simulink library "halin"  (R2021b)
settings: Solver=VariableStepAuto  StartTime=0.0  StopTime=10.0  RelTol=1e-3
undefined symbols (not defined in the file): KHAL_CAN1ABM1E2E_flg, KHAL_CAN1EPB1E2E_flg, KHAL_CAN1EPS1E2E_flg, KHAL_CAN1ESC1E2E_flg, KHAL_CAN1ESC5E2E_flg, KHAL_CAN3BMS1E2E_flg, KHAL_CAN3BMS6E2E_flg, KHAL_CAN3CCU1E2E_flg, KHAL_CAN3CCU2E2E_flg, KHAL_CAN3MCUBF1E2E_flg, KHAL_CAN3MCUBR1E2E_flg, KHAL_CAN3MCUNF1E2E_flg, KHAL_CAN3MCUNR1E2E_flg, KHAL_CAN3Shifter1E2E_flg, KHAL_CAN3Shifter2E2E_flg, KHAL_CAN6FCM2E2E_flg, KHAL_CAN6FCM4E2E_flg, TRUE
libraries: simulink x791, FVT_lib x214, hcu_lib x58
(part 3 of 25)

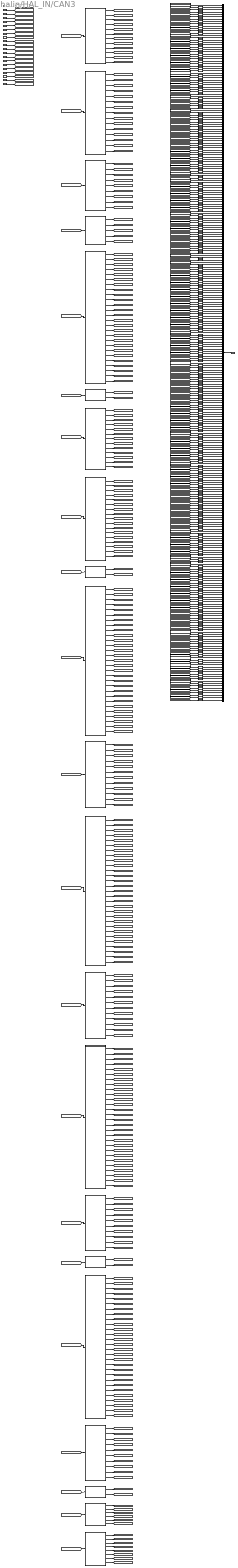
== system halin/HAL_IN/CAN3 ==
  DT_CAN3_SG_BMS1 : Inport
  DT_CAN3_SG_BMS3 : Inport  Port=2
  DT_CAN3_SG_BMS4 : Inport  Port=3
  DT_CAN3_SG_BMS5 : Inport  Port=4
  DT_CAN3_SG_BMS6 : Inport  Port=5
  DT_CAN3_SG_BMS8 : Inport  Port=6
  DT_CAN3_SG_CCU1 : Inport  Port=7
  DT_CAN3_SG_CCU2 : Inport  Port=8
  DT_CAN3_SG_EBM1 : Inport  Port=9
  DT_CAN3_SG_MCU_B_F1 : Inport  Port=10
  DT_CAN3_SG_MCU_B_F2 : Inport  Port=11
  DT_CAN3_SG_MCU_B_R1 : Inport  Port=12
  DT_CAN3_SG_MCU_B_R2 : Inport  Port=13
  DT_CAN3_SG_MCU_N_F1 : Inport  Port=14
  DT_CAN3_SG_MCU_N_F2 : Inport  Port=15
  DT_CAN3_SG_MCU_N_F3 : Inport  Port=16
  DT_CAN3_SG_MCU_N_R1 : Inport  Port=17
  DT_CAN3_SG_MCU_N_R2 : Inport  Port=18
  DT_CAN3_SG_MCU_N_R3 : Inport  Port=19
  DT_CAN3_SG_Shifter1 : Inport  Port=20
  DT_CAN3_SG_Shifter2 : Inport  Port=21
  BMS1 : Subsystem
  BMS3 : Subsystem
  BMS4 : Subsystem
  BMS5 : Subsystem
  BMS6 : Subsystem
  BMS8 : Subsystem
  CCU1 : Subsystem
  CCU2 : Subsystem
  EBM1 : Subsystem
  MCU_B_F1 : Subsystem
  MCU_B_F2 : Subsystem
  MCU_B_R1 : Subsystem
  MCU_B_R2 : Subsystem
  MCU_N_F1 : Subsystem
  MCU_N_F2 : Subsystem
  MCU_N_F3 : Subsystem
  MCU_N_R1 : Subsystem
  MCU_N_R2 : Subsystem
  MCU_N_R3 : Subsystem
  Shifter1 : Subsystem
  Shifter2 : Subsystem
  UnitConverter{,1,13,22,41..42,45..53,59..61,65,69..70,80,82..83,85,87,91,93..94,101..105,114..115,117..119,142..143,146..148,157..158,160..162,183..187,196..197,199..201,223..224,226..228,237..238,240..242,263..264,269..271,274} (75 alike) : DataTypeConversion  OutDataTypeStr=boolean
  UnitConverter{4..12,14..21,23..31,36..40,72..75,77..78,88..90,95,106,108,111..113,121..127,129..130,135..136,145,149,151,154..156,164..170,172,177..178,188,190,193..195,203..209,211..212,217..218,229,231,234..236,244..252,257..258} (105 alike) : DataTypeConversion  OutDataTypeStr=single
  UnitConverter{2..3,32..35,43..44,54..58,62..64,66..68,71,76,79,81,84,86,92,96..100,107,109..110,116,120,128,131..134,137,140..141,144,150,152..153,159,163,171,173..176,181..182,189,191..192,198,202,210,213..216,219..220,225,230,232..233,239,243,253..256,259..260,265..268,272..273,275..276} (89 alike) : DataTypeConversion  OutDataTypeStr=uint8
  UnitConverter{138..139,179..180,221..222,261..262} (8 alike) : DataTypeConversion  OutDataTypeStr=uint16
  VHAL_CANMsgInvalidBMS1_flg : Subsystem  AncestorBlock=FVT_lib/hal/MsgTimeoutJudge_CAN_AUTOSAR
      mask help: MeasumentTrigerEvent
      mask Display: fprintf('MsgTimeoutJudge_CAN\nAUTOSAR');
  VHAL_CANMsgInvalidBMS3_flg : Subsystem  AncestorBlock=FVT_lib/hal/MsgTimeoutJudge_CAN_AUTOSAR
      mask help: MeasumentTrigerEvent
      mask Display: fprintf('MsgTimeoutJudge_CAN\nAUTOSAR');
  VHAL_CANMsgInvalidBMS4_flg : Subsystem  AncestorBlock=FVT_lib/hal/MsgTimeoutJudge_CAN_AUTOSAR
      mask help: MeasumentTrigerEvent
      mask Display: fprintf('MsgTimeoutJudge_CAN\nAUTOSAR');
  VHAL_CANMsgInvalidBMS5_flg : Subsystem  AncestorBlock=FVT_lib/hal/MsgTimeoutJudge_CAN_AUTOSAR
      mask help: MeasumentTrigerEvent
      mask Display: fprintf('MsgTimeoutJudge_CAN\nAUTOSAR');
  VHAL_CANMsgInvalidBMS6_flg : Subsystem  AncestorBlock=FVT_lib/hal/MsgTimeoutJudge_CAN_AUTOSAR
      mask help: MeasumentTrigerEvent
      mask Display: fprintf('MsgTimeoutJudge_CAN\nAUTOSAR');
  VHAL_CANMsgInvalidBMS8_flg : Subsystem  AncestorBlock=FVT_lib/hal/MsgTimeoutJudge_CAN_AUTOSAR
      mask help: MeasumentTrigerEvent
      mask Display: fprintf('MsgTimeoutJudge_CAN\nAUTOSAR');
  VHAL_CANMsgInvalidCCU1_flg : Subsystem  AncestorBlock=FVT_lib/hal/MsgTimeoutJudge_CAN_AUTOSAR
      mask help: MeasumentTrigerEvent
      mask Display: fprintf('MsgTimeoutJudge_CAN\nAUTOSAR');
  VHAL_CANMsgInvalidCCU2_flg : Subsystem  AncestorBlock=FVT_lib/hal/MsgTimeoutJudge_CAN_AUTOSAR
      mask help: MeasumentTrigerEvent
      mask Display: fprintf('MsgTimeoutJudge_CAN\nAUTOSAR');
  VHAL_CANMsgInvalidEBM1_flg : Subsystem  AncestorBlock=FVT_lib/hal/MsgTimeoutJudge_CAN_AUTOSAR
      mask help: MeasumentTrigerEvent
      mask Display: fprintf('MsgTimeoutJudge_CAN\nAUTOSAR');
  VHAL_CANMsgInvalidMCUBF1_flg : Subsystem  AncestorBlock=FVT_lib/hal/MsgTimeoutJudge_CAN_AUTOSAR
      mask help: MeasumentTrigerEvent
      mask Display: fprintf('MsgTimeoutJudge_CAN\nAUTOSAR');
  VHAL_CANMsgInvalidMCUBF2_flg : Subsystem  AncestorBlock=FVT_lib/hal/MsgTimeoutJudge_CAN_AUTOSAR
      mask help: MeasumentTrigerEvent
      mask Display: fprintf('MsgTimeoutJudge_CAN\nAUTOSAR');
  VHAL_CANMsgInvalidMCUBR1_flg : Subsystem  AncestorBlock=FVT_lib/hal/MsgTimeoutJudge_CAN_AUTOSAR
      mask help: MeasumentTrigerEvent
      mask Display: fprintf('MsgTimeoutJudge_CAN\nAUTOSAR');
  VHAL_CANMsgInvalidMCUBR2_flg : Subsystem  AncestorBlock=FVT_lib/hal/MsgTimeoutJudge_CAN_AUTOSAR
      mask help: MeasumentTrigerEvent
      mask Display: fprintf('MsgTimeoutJudge_CAN\nAUTOSAR');
  VHAL_CANMsgInvalidMCUNF1_flg : Subsystem  AncestorBlock=FVT_lib/hal/MsgTimeoutJudge_CAN_AUTOSAR
      mask help: MeasumentTrigerEvent
      mask Display: fprintf('MsgTimeoutJudge_CAN\nAUTOSAR');
  VHAL_CANMsgInvalidMCUNF2_flg : Subsystem  AncestorBlock=FVT_lib/hal/MsgTimeoutJudge_CAN_AUTOSAR
      mask help: MeasumentTrigerEvent
      mask Display: fprintf('MsgTimeoutJudge_CAN\nAUTOSAR');
  VHAL_CANMsgInvalidMCUNF3_flg : Subsystem  AncestorBlock=FVT_lib/hal/MsgTimeoutJudge_CAN_AUTOSAR
      mask help: MeasumentTrigerEvent
      mask Display: fprintf('MsgTimeoutJudge_CAN\nAUTOSAR');
  VHAL_CANMsgInvalidMCUNR1_flg : Subsystem  AncestorBlock=FVT_lib/hal/MsgTimeoutJudge_CAN_AUTOSAR
      mask help: MeasumentTrigerEvent
      mask Display: fprintf('MsgTimeoutJudge_CAN\nAUTOSAR');
  VHAL_CANMsgInvalidMCUNR2_flg : Subsystem  AncestorBlock=FVT_lib/hal/MsgTimeoutJudge_CAN_AUTOSAR
      mask help: MeasumentTrigerEvent
      mask Display: fprintf('MsgTimeoutJudge_CAN\nAUTOSAR');
  VHAL_CANMsgInvalidMCUNR3_flg : Subsystem  AncestorBlock=FVT_lib/hal/MsgTimeoutJudge_CAN_AUTOSAR
      mask help: MeasumentTrigerEvent
      mask Display: fprintf('MsgTimeoutJudge_CAN\nAUTOSAR');
  VHAL_CANMsgInvalidShifter1_flg : Subsystem  AncestorBlock=FVT_lib/hal/MsgTimeoutJudge_CAN_AUTOSAR
      mask help: MeasumentTrigerEvent
      mask Display: fprintf('MsgTimeoutJudge_CAN\nAUTOSAR');
  VHAL_CANMsgInvalidShifter2_flg : Subsystem  AncestorBlock=FVT_lib/hal/MsgTimeoutJudge_CAN_AUTOSAR
      mask help: MeasumentTrigerEvent
      mask Display: fprintf('MsgTimeoutJudge_CAN\nAUTOSAR');
  bus_creator : BusCreator  Inputs=298  OutDataTypeStr=Bus: BHAL_CAN3_outputs  NonVirtualBus=on
  HAL_CAN3_outputs : Outport
  wires:
  DT_CAN3_SG_BMS1/1 -> [DT_CAN3_SG_BMS1]
  DT_CAN3_SG_BMS3/1 -> [DT_CAN3_SG_BMS3]
  DT_CAN3_SG_BMS4/1 -> [DT_CAN3_SG_BMS4]
  DT_CAN3_SG_BMS5/1 -> [DT_CAN3_SG_BMS5]
  DT_CAN3_SG_BMS6/1 -> [DT_CAN3_SG_BMS6]
  DT_CAN3_SG_BMS8/1 -> [DT_CAN3_SG_BMS8]
  DT_CAN3_SG_CCU1/1 -> [DT_CAN3_SG_CCU1]
  DT_CAN3_SG_CCU2/1 -> [DT_CAN3_SG_CCU2]
  DT_CAN3_SG_EBM1/1 -> [DT_CAN3_SG_EBM1]
  DT_CAN3_SG_MCU_B_F1/1 -> [DT_CAN3_SG_MCU_B_F1]
  DT_CAN3_SG_MCU_B_F2/1 -> [DT_CAN3_SG_MCU_B_F2]
  DT_CAN3_SG_MCU_B_R1/1 -> [DT_CAN3_SG_MCU_B_R1]
  DT_CAN3_SG_MCU_B_R2/1 -> [DT_CAN3_SG_MCU_B_R2]
  DT_CAN3_SG_MCU_N_F1/1 -> [DT_CAN3_SG_MCU_N_F1]
  DT_CAN3_SG_MCU_N_F2/1 -> [DT_CAN3_SG_MCU_N_F2]
  DT_CAN3_SG_MCU_N_F3/1 -> [DT_CAN3_SG_MCU_N_F3]
  DT_CAN3_SG_MCU_N_R1/1 -> [DT_CAN3_SG_MCU_N_R1]
  DT_CAN3_SG_MCU_N_R2/1 -> [DT_CAN3_SG_MCU_N_R2]
  DT_CAN3_SG_MCU_N_R3/1 -> [DT_CAN3_SG_MCU_N_R3]
  DT_CAN3_SG_Shifter1/1 -> [DT_CAN3_SG_Shifter1]
  DT_CAN3_SG_Shifter2/1 -> [DT_CAN3_SG_Shifter2]
  [DT_CAN3_SG_BMS1] -> BMS1/1(DT_CAN3_SG_BMS1)
  [DT_CAN3_SG_BMS3] -> BMS3/1(DT_CAN3_SG_BMS3)
  [DT_CAN3_SG_BMS4] -> BMS4/1(DT_CAN3_SG_BMS4)
  [DT_CAN3_SG_BMS5] -> BMS5/1(DT_CAN3_SG_BMS5)
  [DT_CAN3_SG_BMS6] -> BMS6/1(DT_CAN3_SG_BMS6)
  [DT_CAN3_SG_BMS8] -> BMS8/1(DT_CAN3_SG_BMS8)
  [DT_CAN3_SG_CCU1] -> CCU1/1(DT_CAN3_SG_CCU1)
  [DT_CAN3_SG_CCU2] -> CCU2/1(DT_CAN3_SG_CCU2)
  [DT_CAN3_SG_EBM1] -> EBM1/1(DT_CAN3_SG_EBM1)
  [DT_CAN3_SG_MCU_B_F1] -> MCU_B_F1/1(DT_CAN3_SG_MCU_B_F1)
  [DT_CAN3_SG_MCU_B_F2] -> MCU_B_F2/1(DT_CAN3_SG_MCU_B_F2)
  [DT_CAN3_SG_MCU_B_R1] -> MCU_B_R1/1(DT_CAN3_SG_MCU_B_R1)
  [DT_CAN3_SG_MCU_B_R2] -> MCU_B_R2/1(DT_CAN3_SG_MCU_B_R2)
  [DT_CAN3_SG_MCU_N_F1] -> MCU_N_F1/1(DT_CAN3_SG_MCU_N_F1)
  [DT_CAN3_SG_MCU_N_F2] -> MCU_N_F2/1(DT_CAN3_SG_MCU_N_F2)
  [DT_CAN3_SG_MCU_N_F3] -> MCU_N_F3/1(DT_CAN3_SG_MCU_N_F3)
  [DT_CAN3_SG_MCU_N_R1] -> MCU_N_R1/1(DT_CAN3_SG_MCU_N_R1)
  [DT_CAN3_SG_MCU_N_R2] -> MCU_N_R2/1(DT_CAN3_SG_MCU_N_R2)
  [DT_CAN3_SG_MCU_N_R3] -> MCU_N_R3/1(DT_CAN3_SG_MCU_N_R3)
  [DT_CAN3_SG_Shifter1] -> Shifter1/1(DT_CAN3_SG_Shifter1)
  [DT_CAN3_SG_Shifter2] -> Shifter2/1(DT_CAN3_SG_Shifter2)
  bus_creator/1 -> HAL_CAN3_outputs/1
  VHAL_CANMsgInvalidBMS1_flg/1(Out) -> bus_creator/1
  BMS1/1(VHAL_BMS1CSErr_flg) -> [VHAL_BMS1CSErr_flg]
  UnitConverter/1 -> bus_creator/2  "VHAL_BMS1CSErr_flg"
  [VHAL_BMS1CSErr_flg] -> UnitConverter/1
  BMS1/2(VHAL_BMS1RCErr_flg) -> [VHAL_BMS1RCErr_flg]
  UnitConverter1/1 -> bus_creator/3  "VHAL_BMS1RCErr_flg"
  [VHAL_BMS1RCErr_flg] -> UnitConverter1/1
  BMS1/3(VHAL_BMSChckSum1_enum) -> [VHAL_BMSChckSum1_enum]
  UnitConverter2/1 -> bus_creator/4  "VHAL_BMSChckSum1_enum"
  [VHAL_BMSChckSum1_enum] -> UnitConverter2/1
  BMS1/4(VHAL_BMSRolCnct1_enum) -> [VHAL_BMSRolCnct1_enum]
  UnitConverter3/1 -> bus_creator/5  "VHAL_BMSRolCnct1_enum"
  [VHAL_BMSRolCnct1_enum] -> UnitConverter3/1
  BMS1/5(VHAL_HVBPwrAvailChrg_kW) -> [VHAL_HVBPwrAvailChrg_kW]
  UnitConverter4/1 -> bus_creator/6  "VHAL_HVBPwrAvailChrg_kW"
  [VHAL_HVBPwrAvailChrg_kW] -> UnitConverter4/1
  BMS1/6(VHAL_HVBPwrAvailChrg30_kW) -> [VHAL_HVBPwrAvailChrg30_kW]
  UnitConverter5/1 -> bus_creator/7  "VHAL_HVBPwrAvailChrg30_kW"
  [VHAL_HVBPwrAvailChrg30_kW] -> UnitConverter5/1
  BMS1/7(VHAL_HVBPwrAvailChrg60_kW) -> [VHAL_HVBPwrAvailChrg60_kW]
  UnitConverter6/1 -> bus_creator/8  "VHAL_HVBPwrAvailChrg60_kW"
  [VHAL_HVBPwrAvailChrg60_kW] -> UnitConverter6/1
  BMS1/8(VHAL_HVBPwrAvailDchrg_kW) -> [VHAL_HVBPwrAvailDchrg_kW]
  UnitConverter7/1 -> bus_creator/9  "VHAL_HVBPwrAvailDchrg_kW"
  [VHAL_HVBPwrAvailDchrg_kW] -> UnitConverter7/1
  BMS1/9(VHAL_HVBPwrAvailDchrg30_kW) -> [VHAL_HVBPwrAvailDchrg30_kW]
  UnitConverter8/1 -> bus_creator/10  "VHAL_HVBPwrAvailDchrg30_kW"
  [VHAL_HVBPwrAvailDchrg30_kW] -> UnitConverter8/1
  BMS1/10(VHAL_HVBPwrAvailDchrg60_kW) -> [VHAL_HVBPwrAvailDchrg60_kW]
  UnitConverter9/1 -> bus_creator/11  "VHAL_HVBPwrAvailDchrg60_kW"
  [VHAL_HVBPwrAvailDchrg60_kW] -> UnitConverter9/1
  BMS1/11(VHAL_HVBattCurr_A) -> [VHAL_HVBattCurr_A]
  UnitConverter10/1 -> bus_creator/12  "VHAL_HVBattCurr_A"
  [VHAL_HVBattCurr_A] -> UnitConverter10/1
  BMS1/12(VHAL_HVBattVolt_V) -> [VHAL_HVBattVolt_V]
  UnitConverter11/1 -> bus_creator/13  "VHAL_HVBattVolt_V"
  [VHAL_HVBattVolt_V] -> UnitConverter11/1
  VHAL_CANMsgInvalidBMS3_flg/1(Out) -> bus_creator/14
  BMS3/1(VHAL_ACChrgCurrDis_A) -> [VHAL_ACChrgCurrDis_A]
  UnitConverter12/1 -> bus_creator/15  "VHAL_ACChrgCurrDis_A"
  [VHAL_ACChrgCurrDis_A] -> UnitConverter12/1
  BMS3/2(VHAL_FireDetErr_flg) -> [VHAL_FireDetErr_flg]
  UnitConverter13/1 -> bus_creator/16  "VHAL_FireDetErr_flg"
  [VHAL_FireDetErr_flg] -> UnitConverter13/1
  BMS3/3(VHAL_HVBChrgPwr_kWh) -> [VHAL_HVBChrgPwr_kWh]
  UnitConverter14/1 -> bus_creator/17  "VHAL_HVBChrgPwr_kWh"
  [VHAL_HVBChrgPwr_kWh] -> UnitConverter14/1
  BMS3/4(VHAL_HVBChrgPwrTotal_kWh) -> [VHAL_HVBChrgPwrTotal_kWh]
  UnitConverter15/1 -> bus_creator/18  "VHAL_HVBChrgPwrTotal_kWh"
  [VHAL_HVBChrgPwrTotal_kWh] -> UnitConverter15/1
  BMS3/5(VHAL_HVBDrvPwr_kWh) -> [VHAL_HVBDrvPwr_kWh]
  UnitConverter16/1 -> bus_creator/19  "VHAL_HVBDrvPwr_kWh"
  [VHAL_HVBDrvPwr_kWh] -> UnitConverter16/1
  BMS3/6(VHAL_HVBDrvPwrTotal_kWh) -> [VHAL_HVBDrvPwrTotal_kWh]
  UnitConverter17/1 -> bus_creator/20  "VHAL_HVBDrvPwrTotal_kWh"
  [VHAL_HVBDrvPwrTotal_kWh] -> UnitConverter17/1
  BMS3/7(VHAL_HVBFullChrgPwr_kWh) -> [VHAL_HVBFullChrgPwr_kWh]
  UnitConverter18/1 -> bus_creator/21  "VHAL_HVBFullChrgPwr_kWh"
  [VHAL_HVBFullChrgPwr_kWh] -> UnitConverter18/1
  BMS3/8(VHAL_HVBIsoImpedenceN_Megaohm) -> [VHAL_HVBIsoImpedenceN_Megaohm]
  UnitConverter19/1 -> bus_creator/22  "VHAL_HVBIsoImpedenceN_Megaohm"
  [VHAL_HVBIsoImpedenceN_Megaohm] -> UnitConverter19/1
  BMS3/9(VHAL_HVBIsoImpedenceP_Megaohm) -> [VHAL_HVBIsoImpedenceP_Megaohm]
  UnitConverter20/1 -> bus_creator/23  "VHAL_HVBIsoImpedenceP_Megaohm"
  [VHAL_HVBIsoImpedenceP_Megaohm] -> UnitConverter20/1
  BMS3/10(VHAL_HVBSOH_pct) -> [VHAL_HVBSOH_pct]
  UnitConverter21/1 -> bus_creator/24  "VHAL_HVBSOH_pct"
  [VHAL_HVBSOH_pct] -> UnitConverter21/1
  BMS3/11(VHAL_HVBattErr_flg) -> [VHAL_HVBattErr_flg]
  UnitConverter22/1 -> bus_creator/25  "VHAL_HVBattErr_flg"
  [VHAL_HVBattErr_flg] -> UnitConverter22/1
  BMS3/12(VHAL_HVBattPackVolt_V) -> [VHAL_HVBattPackVolt_V]
  UnitConverter23/1 -> bus_creator/26  "VHAL_HVBattPackVolt_V"
  [VHAL_HVBattPackVolt_V] -> UnitConverter23/1
  BMS3/13(VHAL_HVBattSOC_pct) -> [VHAL_HVBattSOC_pct]
  UnitConverter24/1 -> bus_creator/27  "VHAL_HVBattSOC_pct"
  [VHAL_HVBattSOC_pct] -> UnitConverter24/1
  BMS3/14(VHAL_HVBattSOCDis_pct) -> [VHAL_HVBattSOCDis_pct]
  UnitConverter25/1 -> bus_creator/28  "VHAL_HVBattSOCDis_pct"
  [VHAL_HVBattSOCDis_pct] -> UnitConverter25/1
  BMS3/15(VHAL_RemainChrgTime_min) -> [VHAL_RemainChrgTime_min]
  UnitConverter26/1 -> bus_creator/29  "VHAL_RemainChrgTime_min"
  [VHAL_RemainChrgTime_min] -> UnitConverter26/1
  VHAL_CANMsgInvalidBMS4_flg/1(Out) -> bus_creator/30
  BMS4/1(VHAL_CellTempAvg_C) -> [VHAL_CellTempAvg_C]
  UnitConverter27/1 -> bus_creator/31  "VHAL_CellTempAvg_C"
  [VHAL_CellTempAvg_C] -> UnitConverter27/1
  BMS4/2(VHAL_HVBCellVoltMax_mV) -> [VHAL_HVBCellVoltMax_mV]
  UnitConverter28/1 -> bus_creator/32  "VHAL_HVBCellVoltMax_mV"
  [VHAL_HVBCellVoltMax_mV] -> UnitConverter28/1
  BMS4/3(VHAL_HVBCellVoltMin_mV) -> [VHAL_HVBCellVoltMin_mV]
  UnitConverter29/1 -> bus_creator/33  "VHAL_HVBCellVoltMin_mV"
  [VHAL_HVBCellVoltMin_mV] -> UnitConverter29/1
  BMS4/4(VHAL_HVBMTempMax_C) -> [VHAL_HVBMTempMax_C]
  UnitConverter30/1 -> bus_creator/34  "VHAL_HVBMTempMax_C"
  [VHAL_HVBMTempMax_C] -> UnitConverter30/1
  BMS4/5(VHAL_HVBMTempMin_C) -> [VHAL_HVBMTempMin_C]
  UnitConverter31/1 -> bus_creator/35  "VHAL_HVBMTempMin_C"
  [VHAL_HVBMTempMin_C] -> UnitConverter31/1
  BMS4/6(VHAL_MaxCellTempNum_enum) -> [VHAL_MaxCellTempNum_enum]
  UnitConverter32/1 -> bus_creator/36  "VHAL_MaxCellTempNum_enum"
  [VHAL_MaxCellTempNum_enum] -> UnitConverter32/1
  BMS4/7(VHAL_MaxCellVoltNum_enum) -> [VHAL_MaxCellVoltNum_enum]
  UnitConverter33/1 -> bus_creator/37  "VHAL_MaxCellVoltNum_enum"
  [VHAL_MaxCellVoltNum_enum] -> UnitConverter33/1
  BMS4/8(VHAL_MinCellTempNum_enum) -> [VHAL_MinCellTempNum_enum]
  UnitConverter34/1 -> bus_creator/38  "VHAL_MinCellTempNum_enum"
  [VHAL_MinCellTempNum_enum] -> UnitConverter34/1
  BMS4/9(VHAL_MinCellVoltNum_enum) -> [VHAL_MinCellVoltNum_enum]
  UnitConverter35/1 -> bus_creator/39  "VHAL_MinCellVoltNum_enum"
  [VHAL_MinCellVoltNum_enum] -> UnitConverter35/1
  VHAL_CANMsgInvalidBMS5_flg/1(Out) -> bus_creator/40
  BMS5/1(VHAL_HVInVolt_V) -> [VHAL_HVInVolt_V]
  UnitConverter36/1 -> bus_creator/41  "VHAL_HVInVolt_V"
  [VHAL_HVInVolt_V] -> UnitConverter36/1
  BMS5/2(VHAL_LVBattDet12V_V) -> [VHAL_LVBattDet12V_V]
  UnitConverter37/1 -> bus_creator/42  "VHAL_LVBattDet12V_V"
  [VHAL_LVBattDet12V_V] -> UnitConverter37/1
  BMS5/3(VHAL_OBCACCSLimit_A) -> [VHAL_OBCACCSLimit_A]
  UnitConverter38/1 -> bus_creator/43  "VHAL_OBCACCSLimit_A"
  [VHAL_OBCACCSLimit_A] -> UnitConverter38/1
  BMS5/4(VHAL_OBCDCCurLm_A) -> [VHAL_OBCDCCurLm_A]
  UnitConverter39/1 -> bus_creator/44  "VHAL_OBCDCCurLm_A"
  [VHAL_OBCDCCurLm_A] -> UnitConverter39/1
  BMS5/5(VHAL_OBCDCVoltLm_V) -> [VHAL_OBCDCVoltLm_V]
  UnitConverter40/1 -> bus_creator/45  "VHAL_OBCDCVoltLm_V"
  [VHAL_OBCDCVoltLm_V] -> UnitConverter40/1
  VHAL_CANMsgInvalidBMS6_flg/1(Out) -> bus_creator/46
  BMS6/1(VHAL_BMS6CSErr_flg) -> [VHAL_BMS6CSErr_flg]
  UnitConverter41/1 -> bus_creator/47  "VHAL_BMS6CSErr_flg"
  [VHAL_BMS6CSErr_flg] -> UnitConverter41/1
  BMS6/2(VHAL_BMS6RCErr_flg) -> [VHAL_BMS6RCErr_flg]
  UnitConverter42/1 -> bus_creator/48  "VHAL_BMS6RCErr_flg"
  [VHAL_BMS6RCErr_flg] -> UnitConverter42/1
  BMS6/3(VHAL_BMSChckSum_enum) -> [VHAL_BMSChckSum_enum]
  UnitConverter43/1 -> bus_creator/49  "VHAL_BMSChckSum_enum"
  [VHAL_BMSChckSum_enum] -> UnitConverter43/1
  BMS6/4(VHAL_BMSRolCnct_enum) -> [VHAL_BMSRolCnct_enum]
  UnitConverter44/1 -> bus_creator/50  "VHAL_BMSRolCnct_enum"
  [VHAL_BMSRolCnct_enum] -> UnitConverter44/1
  BMS6/5(VHAL_BMSREADY_flg) -> [VHAL_BMSREADY_flg]
  UnitConverter45/1 -> bus_creator/51  "VHAL_BMSREADY_flg"
  [VHAL_BMSREADY_flg] -> UnitConverter45/1
  BMS6/6(VHAL_BMSWarn1_flg) -> [VHAL_BMSWarn1_flg]
  UnitConverter46/1 -> bus_creator/52  "VHAL_BMSWarn1_flg"
  [VHAL_BMSWarn1_flg] -> UnitConverter46/1
  BMS6/7(VHAL_BMSWarn2_flg) -> [VHAL_BMSWarn2_flg]
  UnitConverter47/1 -> bus_creator/53  "VHAL_BMSWarn2_flg"
  [VHAL_BMSWarn2_flg] -> UnitConverter47/1
  BMS6/8(VHAL_BMSWarn3_flg) -> [VHAL_BMSWarn3_flg]
  UnitConverter48/1 -> bus_creator/54  "VHAL_BMSWarn3_flg"
  [VHAL_BMSWarn3_flg] -> UnitConverter48/1
  BMS6/9(VHAL_BMSWarn4_flg) -> [VHAL_BMSWarn4_flg]
  UnitConverter49/1 -> bus_creator/55  "VHAL_BMSWarn4_flg"
  [VHAL_BMSWarn4_flg] -> UnitConverter49/1
  BMS6/10(VHAL_BMSWarn5_flg) -> [VHAL_BMSWarn5_flg]
  UnitConverter50/1 -> bus_creator/56  "VHAL_BMSWarn5_flg"
  [VHAL_BMSWarn5_flg] -> UnitConverter50/1
  BMS6/11(VHAL_BMSWarn6_flg) -> [VHAL_BMSWarn6_flg]
  UnitConverter51/1 -> bus_creator/57  "VHAL_BMSWarn6_flg"
  [VHAL_BMSWarn6_flg] -> UnitConverter51/1
  BMS6/12(VHAL_BMSWarn7_flg) -> [VHAL_BMSWarn7_flg]
  UnitConverter52/1 -> bus_creator/58  "VHAL_BMSWarn7_flg"
  [VHAL_BMSWarn7_flg] -> UnitConverter52/1
  BMS6/13(VHAL_BMSWarn8_flg) -> [VHAL_BMSWarn8_flg]
  UnitConverter53/1 -> bus_creator/59  "VHAL_BMSWarn8_flg"
  [VHAL_BMSWarn8_flg] -> UnitConverter53/1
  BMS6/14(VHAL_ChrgInLockReq_enum) -> [VHAL_ChrgInLockReq_enum]
  UnitConverter54/1 -> bus_creator/60  "VHAL_ChrgInLockReq_enum"
  [VHAL_ChrgInLockReq_enum] -> UnitConverter54/1
  BMS6/15(VHAL_ChrgPlugSta_enum) -> [VHAL_ChrgPlugSta_enum]
  UnitConverter55/1 -> bus_creator/61  "VHAL_ChrgPlugSta_enum"
  [VHAL_ChrgPlugSta_enum] -> UnitConverter55/1
  BMS6/16(VHAL_DisChrgPlugErr_enum) -> [VHAL_DisChrgPlugErr_enum]
  UnitConverter56/1 -> bus_creator/62  "VHAL_DisChrgPlugErr_enum"
  [VHAL_DisChrgPlugErr_enum] -> UnitConverter56/1
  BMS6/17(VHAL_ExtChrgSta_enum) -> [VHAL_ExtChrgSta_enum]
  UnitConverter57/1 -> bus_creator/63  "VHAL_ExtChrgSta_enum"
  [VHAL_ExtChrgSta_enum] -> UnitConverter57/1
  BMS6/18(VHAL_HVBChrgErr_enum) -> [VHAL_HVBChrgErr_enum]
  UnitConverter58/1 -> bus_creator/64  "VHAL_HVBChrgErr_enum"
  [VHAL_HVBChrgErr_enum] -> UnitConverter58/1
  BMS6/19(VHAL_HVBContactorSta_flg) -> [VHAL_HVBContactorSta_flg]
  UnitConverter59/1 -> bus_creator/65  "VHAL_HVBContactorSta_flg"
  [VHAL_HVBContactorSta_flg] -> UnitConverter59/1
  BMS6/20(VHAL_HVBHVILErr_flg) -> [VHAL_HVBHVILErr_flg]
  UnitConverter60/1 -> bus_creator/66  "VHAL_HVBHVILErr_flg"
  [VHAL_HVBHVILErr_flg] -> UnitConverter60/1
  BMS6/21(VHAL_HVBOvrTempErr_flg) -> [VHAL_HVBOvrTempErr_flg]
  UnitConverter61/1 -> bus_creator/67  "VHAL_HVBOvrTempErr_flg"
  [VHAL_HVBOvrTempErr_flg] -> UnitConverter61/1
  BMS6/22(VHAL_HVBOvrTempWarn_enum) -> [VHAL_HVBOvrTempWarn_enum]
  UnitConverter62/1 -> bus_creator/68  "VHAL_HVBOvrTempWarn_enum"
  [VHAL_HVBOvrTempWarn_enum] -> UnitConverter62/1
  BMS6/23(VHAL_HVBPreheatPrecoolSta_enum) -> [VHAL_HVBPreheatPrecoolSta_enum]
  UnitConverter63/1 -> bus_creator/69  "VHAL_HVBPreheatPrecoolSta_enum"
  [VHAL_HVBPreheatPrecoolSta_enum] -> UnitConverter63/1
  BMS6/24(VHAL_HVBattReady4Pre_enum) -> [VHAL_HVBattReady4Pre_enum]
  UnitConverter64/1 -> bus_creator/70  "VHAL_HVBattReady4Pre_enum"
  [VHAL_HVBattReady4Pre_enum] -> UnitConverter64/1
  BMS6/25(VHAL_HVILSta_flg) -> [VHAL_HVILSta_flg]
  UnitConverter65/1 -> bus_creator/71  "VHAL_HVILSta_flg"
  [VHAL_HVILSta_flg] -> UnitConverter65/1
  BMS6/26(VHAL_V2LSta_enum) -> [VHAL_V2LSta_enum]
  UnitConverter66/1 -> bus_creator/72  "VHAL_V2LSta_enum"
  [VHAL_V2LSta_enum] -> UnitConverter66/1
  VHAL_CANMsgInvalidBMS8_flg/1(Out) -> bus_creator/73
  BMS8/1(VHAL_MainRlyNegSta_enum) -> [VHAL_MainRlyNegSta_enum]
  UnitConverter67/1 -> bus_creator/74  "VHAL_MainRlyNegSta_enum"
  [VHAL_MainRlyNegSta_enum] -> UnitConverter67/1
  BMS8/2(VHAL_MainRlyPosSta_enum) -> [VHAL_MainRlyPosSta_enum]
  UnitConverter68/1 -> bus_creator/75  "VHAL_MainRlyPosSta_enum"
  [VHAL_MainRlyPosSta_enum] -> UnitConverter68/1
  VHAL_CANMsgInvalidCCU1_flg/1(Out) -> bus_creator/76
  CCU1/1(VHAL_CCU1CSErr_flg) -> [VHAL_CCU1CSErr_flg]
  UnitConverter69/1 -> bus_creator/77  "VHAL_CCU1CSErr_flg"
  [VHAL_CCU1CSErr_flg] -> UnitConverter69/1
  CCU1/2(VHAL_CCU1RCErr_flg) -> [VHAL_CCU1RCErr_flg]
  UnitConverter70/1 -> bus_creator/78  "VHAL_CCU1RCErr_flg"
  [VHAL_CCU1RCErr_flg] -> UnitConverter70/1
  CCU1/3(VHAL_CSCCU1_enum) -> [VHAL_CSCCU1_enum]
  UnitConverter71/1 -> bus_creator/79  "VHAL_CSCCU1_enum"
  [VHAL_CSCCU1_enum] -> UnitConverter71/1
  CCU1/4(VHAL_DCDCAuxCur_A) -> [VHAL_DCDCAuxCur_A]
  UnitConverter72/1 -> bus_creator/80  "VHAL_DCDCAuxCur_A"
  [VHAL_DCDCAuxCur_A] -> UnitConverter72/1
  CCU1/5(VHAL_DCDCAuxVolt_V) -> [VHAL_DCDCAuxVolt_V]
  UnitConverter73/1 -> bus_creator/81  "VHAL_DCDCAuxVolt_V"
  [VHAL_DCDCAuxVolt_V] -> UnitConverter73/1
  CCU1/6(VHAL_DCDCHVCur_A) -> [VHAL_DCDCHVCur_A]
  UnitConverter74/1 -> bus_creator/82  "VHAL_DCDCHVCur_A"
  [VHAL_DCDCHVCur_A] -> UnitConverter74/1
  CCU1/7(VHAL_DCDCInVoltInf_V) -> [VHAL_DCDCInVoltInf_V]
  UnitConverter75/1 -> bus_creator/83  "VHAL_DCDCInVoltInf_V"
  [VHAL_DCDCInVoltInf_V] -> UnitConverter75/1
  CCU1/8(VHAL_DCDCPreCompleted_enum) -> [VHAL_DCDCPreCompleted_enum]
  UnitConverter76/1 -> bus_creator/84  "VHAL_DCDCPreCompleted_enum"
  [VHAL_DCDCPreCompleted_enum] -> UnitConverter76/1
  CCU1/9(VHAL_OBCDCCurrInf_A) -> [VHAL_OBCDCCurrInf_A]
  UnitConverter77/1 -> bus_creator/85  "VHAL_OBCDCCurrInf_A"
  [VHAL_OBCDCCurrInf_A] -> UnitConverter77/1
  CCU1/10(VHAL_OBCDCVoltInf_V) -> [VHAL_OBCDCVoltInf_V]
  UnitConverter78/1 -> bus_creator/86  "VHAL_OBCDCVoltInf_V"
  [VHAL_OBCDCVoltInf_V] -> UnitConverter78/1
  CCU1/11(VHAL_OBCPreCompleted_enum) -> [VHAL_OBCPreCompleted_enum]
  UnitConverter79/1 -> bus_creator/87  "VHAL_OBCPreCompleted_enum"
  [VHAL_OBCPreCompleted_enum] -> UnitConverter79/1
  CCU1/12(VHAL_OBCWakeup4Plugin_flg) -> [VHAL_OBCWakeup4Plugin_flg]
  UnitConverter80/1 -> bus_creator/88  "VHAL_OBCWakeup4Plugin_flg"
  [VHAL_OBCWakeup4Plugin_flg] -> UnitConverter80/1
  CCU1/13(VHAL_RCCCU1_enum) -> [VHAL_RCCCU1_enum]
  UnitConverter81/1 -> bus_creator/89  "VHAL_RCCCU1_enum"
  [VHAL_RCCCU1_enum] -> UnitConverter81/1
  VHAL_CANMsgInvalidCCU2_flg/1(Out) -> bus_creator/90
  CCU2/1(VHAL_CCU2CSErr_flg) -> [VHAL_CCU2CSErr_flg]
  UnitConverter82/1 -> bus_creator/91  "VHAL_CCU2CSErr_flg"
  [VHAL_CCU2CSErr_flg] -> UnitConverter82/1
  CCU2/2(VHAL_CCU2RCErr_flg) -> [VHAL_CCU2RCErr_flg]
  UnitConverter83/1 -> bus_creator/92  "VHAL_CCU2RCErr_flg"
  [VHAL_CCU2RCErr_flg] -> UnitConverter83/1
  CCU2/3(VHAL_CSCCU2_enum) -> [VHAL_CSCCU2_enum]
  UnitConverter84/1 -> bus_creator/93  "VHAL_CSCCU2_enum"
  [VHAL_CSCCU2_enum] -> UnitConverter84/1
  CCU2/4(VHAL_DCDCEnaSta_flg) -> [VHAL_DCDCEnaSta_flg]
  UnitConverter85/1 -> bus_creator/94  "VHAL_DCDCEnaSta_flg"
  [VHAL_DCDCEnaSta_flg] -> UnitConverter85/1
  CCU2/5(VHAL_DCDCFaultSta_enum) -> [VHAL_DCDCFaultSta_enum]
  UnitConverter86/1 -> bus_creator/95  "VHAL_DCDCFaultSta_enum"
  [VHAL_DCDCFaultSta_enum] -> UnitConverter86/1
  CCU2/6(VHAL_DCDCReady4Pre_flg) -> [VHAL_DCDCReady4Pre_flg]
  UnitConverter87/1 -> bus_creator/96  "VHAL_DCDCReady4Pre_flg"
  [VHAL_DCDCReady4Pre_flg] -> UnitConverter87/1
  CCU2/7(VHAL_DCDCTemp_C) -> [VHAL_DCDCTemp_C]
  UnitConverter88/1 -> bus_creator/97  "VHAL_DCDCTemp_C"
  [VHAL_DCDCTemp_C] -> UnitConverter88/1
  CCU2/8(VHAL_OBCACCurrInf_A) -> [VHAL_OBCACCurrInf_A]
  UnitConverter89/1 -> bus_creator/98  "VHAL_OBCACCurrInf_A"
  [VHAL_OBCACCurrInf_A] -> UnitConverter89/1
  CCU2/9(VHAL_OBCACVoltInf_V) -> [VHAL_OBCACVoltInf_V]
  UnitConverter90/1 -> bus_creator/99  "VHAL_OBCACVoltInf_V"
  [VHAL_OBCACVoltInf_V] -> UnitConverter90/1
  CCU2/10(VHAL_OBCEnaSta_flg) -> [VHAL_OBCEnaSta_flg]
  UnitConverter91/1 -> bus_creator/100  "VHAL_OBCEnaSta_flg"
  [VHAL_OBCEnaSta_flg] -> UnitConverter91/1
  CCU2/11(VHAL_OBCFaultSta_enum) -> [VHAL_OBCFaultSta_enum]
  UnitConverter92/1 -> bus_creator/101  "VHAL_OBCFaultSta_enum"
  [VHAL_OBCFaultSta_enum] -> UnitConverter92/1
  CCU2/12(VHAL_OBCPluginSta_flg) -> [VHAL_OBCPluginSta_flg]
  UnitConverter93/1 -> bus_creator/102  "VHAL_OBCPluginSta_flg"
  [VHAL_OBCPluginSta_flg] -> UnitConverter93/1
  CCU2/13(VHAL_OBCReady4Pre_flg) -> [VHAL_OBCReady4Pre_flg]
  UnitConverter94/1 -> bus_creator/103  "VHAL_OBCReady4Pre_flg"
  [VHAL_OBCReady4Pre_flg] -> UnitConverter94/1
  CCU2/14(VHAL_OBCTemp_C) -> [VHAL_OBCTemp_C]
  UnitConverter95/1 -> bus_creator/104  "VHAL_OBCTemp_C"
  [VHAL_OBCTemp_C] -> UnitConverter95/1
  CCU2/15(VHAL_OBCV2LSta_enum) -> [VHAL_OBCV2LSta_enum]
  UnitConverter96/1 -> bus_creator/105  "VHAL_OBCV2LSta_enum"
  [VHAL_OBCV2LSta_enum] -> UnitConverter96/1
  CCU2/16(VHAL_OBCACCurLim_enum) -> [VHAL_OBCACCurLim_enum]
  UnitConverter97/1 -> bus_creator/106  "VHAL_OBCACCurLim_enum"
  [VHAL_OBCACCurLim_enum] -> UnitConverter97/1
  CCU2/17(VHAL_RCCCU2_enum) -> [VHAL_RCCCU2_enum]
  UnitConverter98/1 -> bus_creator/107  "VHAL_RCCCU2_enum"
  [VHAL_RCCCU2_enum] -> UnitConverter98/1
  VHAL_CANMsgInvalidEBM1_flg/1(Out) -> bus_creator/108
  EBM1/1(VHAL_EBMErrSta_enum) -> [VHAL_EBMErrSta_enum]
  UnitConverter99/1 -> bus_creator/109  "VHAL_EBMErrSta_enum"
  [VHAL_EBMErrSta_enum] -> UnitConverter99/1
  EBM1/2(VHAL_EBMRLampSta_enum) -> [VHAL_EBMRLampSta_enum]
  UnitConverter100/1 -> bus_creator/110  "VHAL_EBMRLampSta_enum"
  [VHAL_EBMRLampSta_enum] -> UnitConverter100/1
  VHAL_CANMsgInvalidMCUBF1_flg/1(Out) -> bus_creator/111
  MCU_B_F1/1(VHAL_MCUBF1CSErr_flg) -> [VHAL_MCUBF1CSErr_flg]
  UnitConverter101/1 -> bus_creator/112  "VHAL_MCUBF1CSErr_flg"
  [VHAL_MCUBF1CSErr_flg] -> UnitConverter101/1
  MCU_B_F1/2(VHAL_MCUBF1RCErr_flg) -> [VHAL_MCUBF1RCErr_flg]
  UnitConverter102/1 -> bus_creator/113  "VHAL_MCUBF1RCErr_flg"
  [VHAL_MCUBF1RCErr_flg] -> UnitConverter102/1
  MCU_B_F1/3(VHAL_FrActvDmpDisabSta_flg) -> [VHAL_FrActvDmpDisabSta_flg]
  UnitConverter103/1 -> bus_creator/114  "VHAL_FrActvDmpDisabSta_flg"
  [VHAL_FrActvDmpDisabSta_flg] -> UnitConverter103/1
  MCU_B_F1/4(VHAL_FrEDUDrtSta_flg) -> [VHAL_FrEDUDrtSta_flg]
  UnitConverter104/1 -> bus_creator/115  "VHAL_FrEDUDrtSta_flg"
  [VHAL_FrEDUDrtSta_flg] -> UnitConverter104/1
  MCU_B_F1/5(VHAL_FrEDUOpratingSta_flg) -> [VHAL_FrEDUOpratingSta_flg]
  UnitConverter105/1 -> bus_creator/116  "VHAL_FrEDUOpratingSta_flg"
  [VHAL_FrEDUOpratingSta_flg] -> UnitConverter105/1
  MCU_B_F1/6(VHAL_FrEDURealTMTq_Nm) -> [VHAL_FrEDURealTMTq_Nm]
  UnitConverter106/1 -> bus_creator/117  "VHAL_FrEDURealTMTq_Nm"
  [VHAL_FrEDURealTMTq_Nm] -> UnitConverter106/1
  MCU_B_F1/7(VHAL_FrEDURotateDirction_enum) -> [VHAL_FrEDURotateDirction_enum]
  UnitConverter107/1 -> bus_creator/118  "VHAL_FrEDURotateDirction_enum"
  [VHAL_FrEDURotateDirction_enum] -> UnitConverter107/1
  MCU_B_F1/8(VHAL_FrEDUTqReqFbk_Nm) -> [VHAL_FrEDUTqReqFbk_Nm]
  UnitConverter108/1 -> bus_creator/119  "VHAL_FrEDUTqReqFbk_Nm"
  [VHAL_FrEDUTqReqFbk_Nm] -> UnitConverter108/1
  MCU_B_F1/9(VHAL_FrMCU1Chksum_enum) -> [VHAL_FrMCU1Chksum_enum]
  UnitConverter109/1 -> bus_creator/120  "VHAL_FrMCU1Chksum_enum"
  [VHAL_FrMCU1Chksum_enum] -> UnitConverter109/1
  MCU_B_F1/10(VHAL_FrMCU1RolCnt_enum) -> [VHAL_FrMCU1RolCnt_enum]
  UnitConverter110/1 -> bus_creator/121  "VHAL_FrMCU1RolCnt_enum"
  [VHAL_FrMCU1RolCnt_enum] -> UnitConverter110/1
  MCU_B_F1/11(VHAL_FrMCUBAT_V) -> [VHAL_FrMCUBAT_V]
  UnitConverter111/1 -> bus_creator/122  "VHAL_FrMCUBAT_V"
  [VHAL_FrMCUBAT_V] -> UnitConverter111/1
  MCU_B_F1/12(VHAL_FrMCUDCBusCurr_A) -> [VHAL_FrMCUDCBusCurr_A]
  UnitConverter112/1 -> bus_creator/123  "VHAL_FrMCUDCBusCurr_A"
  [VHAL_FrMCUDCBusCurr_A] -> UnitConverter112/1
  MCU_B_F1/13(VHAL_FrMCUDCBusVolt_V) -> [VHAL_FrMCUDCBusVolt_V]
  UnitConverter113/1 -> bus_creator/124  "VHAL_FrMCUDCBusVolt_V"
  [VHAL_FrMCUDCBusVolt_V] -> UnitConverter113/1
  MCU_B_F1/14(VHAL_FrMCUDischrgSta_flg) -> [VHAL_FrMCUDischrgSta_flg]
  UnitConverter114/1 -> bus_creator/125  "VHAL_FrMCUDischrgSta_flg"
  [VHAL_FrMCUDischrgSta_flg] -> UnitConverter114/1
  MCU_B_F1/15(VHAL_FrMCUEnaSta_flg) -> [VHAL_FrMCUEnaSta_flg]
  UnitConverter115/1 -> bus_creator/126  "VHAL_FrMCUEnaSta_flg"
  [VHAL_FrMCUEnaSta_flg] -> UnitConverter115/1
  MCU_B_F1/16(VHAL_FrMCUErr_enum) -> [VHAL_FrMCUErr_enum]
  UnitConverter116/1 -> bus_creator/127  "VHAL_FrMCUErr_enum"
  [VHAL_FrMCUErr_enum] -> UnitConverter116/1
  MCU_B_F1/17(VHAL_FrMCUIGNsta_flg) -> [VHAL_FrMCUIGNsta_flg]
  UnitConverter117/1 -> bus_creator/128  "VHAL_FrMCUIGNsta_flg"
  [VHAL_FrMCUIGNsta_flg] -> UnitConverter117/1
  MCU_B_F1/18(VHAL_FrMCUReady_flg) -> [VHAL_FrMCUReady_flg]
  UnitConverter118/1 -> bus_creator/129  "VHAL_FrMCUReady_flg"
  [VHAL_FrMCUReady_flg] -> UnitConverter118/1
  MCU_B_F1/19(VHAL_FrMCUReady4Pre_flg) -> [VHAL_FrMCUReady4Pre_flg]
  UnitConverter119/1 -> bus_creator/130  "VHAL_FrMCUReady4Pre_flg"
  [VHAL_FrMCUReady4Pre_flg] -> UnitConverter119/1
  MCU_B_F1/20(VHAL_FrMCUSysSta_enum) -> [VHAL_FrMCUSysSta_enum]
  UnitConverter120/1 -> bus_creator/131  "VHAL_FrMCUSysSta_enum"
  [VHAL_FrMCUSysSta_enum] -> UnitConverter120/1
  MCU_B_F1/21(VHAL_FrMCUTemp_C) -> [VHAL_FrMCUTemp_C]
  UnitConverter121/1 -> bus_creator/132  "VHAL_FrMCUTemp_C"
  [VHAL_FrMCUTemp_C] -> UnitConverter121/1
  MCU_B_F1/22(VHAL_FrMotorAvailTq_Nm) -> [VHAL_FrMotorAvailTq_Nm]
  UnitConverter122/1 -> bus_creator/133  "VHAL_FrMotorAvailTq_Nm"
  [VHAL_FrMotorAvailTq_Nm] -> UnitConverter122/1
  MCU_B_F1/23(VHAL_FrRegenAvailTq_Nm) -> [VHAL_FrRegenAvailTq_Nm]
  UnitConverter123/1 -> bus_creator/134  "VHAL_FrRegenAvailTq_Nm"
  [VHAL_FrRegenAvailTq_Nm] -> UnitConverter123/1
  MCU_B_F1/24(VHAL_FrTMSpd_rpm) -> [VHAL_FrTMSpd_rpm]
  UnitConverter124/1 -> bus_creator/135  "VHAL_FrTMSpd_rpm"
  [VHAL_FrTMSpd_rpm] -> UnitConverter124/1
  MCU_B_F1/25(VHAL_FrTMTemp_C) -> [VHAL_FrTMTemp_C]
  UnitConverter125/1 -> bus_creator/136  "VHAL_FrTMTemp_C"
  [VHAL_FrTMTemp_C] -> UnitConverter125/1
  MCU_B_F1/26(VHAL_FrTMid_A) -> [VHAL_FrTMid_A]
  UnitConverter126/1 -> bus_creator/137  "VHAL_FrTMid_A"
  [VHAL_FrTMid_A] -> UnitConverter126/1
  MCU_B_F1/27(VHAL_FrTMiq_A) -> [VHAL_FrTMiq_A]
  UnitConverter127/1 -> bus_creator/138  "VHAL_FrTMiq_A"
  [VHAL_FrTMiq_A] -> UnitConverter127/1
  MCU_B_F1/28(VHAL_MCUWarnF_enum) -> [VHAL_MCUWarnF_enum]
  UnitConverter128/1 -> bus_creator/139  "VHAL_MCUWarnF_enum"
  [VHAL_MCUWarnF_enum] -> UnitConverter128/1
  MCU_B_F1/29(VHAL_MCUBFRealPwrKwSta_kW) -> [VHAL_MCUBFRealPwrKwSta_kW]
  UnitConverter129/1 -> bus_creator/140  "VHAL_MCUBFRealPwrKwSta_kW"
  [VHAL_MCUBFRealPwrKwSta_kW] -> UnitConverter129/1
  VHAL_CANMsgInvalidMCUBF2_flg/1(Out) -> bus_creator/141
  MCU_B_F2/1(VHAL_FrCoolanttempReq_C) -> [VHAL_FrCoolanttempReq_C]
  UnitConverter130/1 -> bus_creator/142  "VHAL_FrCoolanttempReq_C"
  [VHAL_FrCoolanttempReq_C] -> UnitConverter130/1
  MCU_B_F2/2(VHAL_FrFailcode1_enum) -> [VHAL_FrFailcode1_enum]
  UnitConverter131/1 -> bus_creator/143  "VHAL_FrFailcode1_enum"
  [VHAL_FrFailcode1_enum] -> UnitConverter131/1
  MCU_B_F2/3(VHAL_FrFailcode2_enum) -> [VHAL_FrFailcode2_enum]
  UnitConverter132/1 -> bus_creator/144  "VHAL_FrFailcode2_enum"
  [VHAL_FrFailcode2_enum] -> UnitConverter132/1
  MCU_B_F2/4(VHAL_FrFailcodehistory1_enum) -> [VHAL_FrFailcodehistory1_enum]
  UnitConverter133/1 -> bus_creator/145  "VHAL_FrFailcodehistory1_enum"
  [VHAL_FrFailcodehistory1_enum] -> UnitConverter133/1
  MCU_B_F2/5(VHAL_FrFailcodehistory2_enum) -> [VHAL_FrFailcodehistory2_enum]
  UnitConverter134/1 -> bus_creator/146  "VHAL_FrFailcodehistory2_enum"
  [VHAL_FrFailcodehistory2_enum] -> UnitConverter134/1
  MCU_B_F2/6(VHAL_FrLLCTemp_C) -> [VHAL_FrLLCTemp_C]
  UnitConverter135/1 -> bus_creator/147  "VHAL_FrLLCTemp_C"
  [VHAL_FrLLCTemp_C] -> UnitConverter135/1
  MCU_B_F2/7(VHAL_FrLLCflowReq_Lpmin) -> [VHAL_FrLLCflowReq_Lpmin]
  UnitConverter136/1 -> bus_creator/148  "VHAL_FrLLCflowReq_Lpmin"
  [VHAL_FrLLCflowReq_Lpmin] -> UnitConverter136/1
  MCU_B_F2/8(VHAL_FrMCUTempWarn_enum) -> [VHAL_FrMCUTempWarn_enum]
  UnitConverter137/1 -> bus_creator/149  "VHAL_FrMCUTempWarn_enum"
  [VHAL_FrMCUTempWarn_enum] -> UnitConverter137/1
  MCU_B_F2/9(VHAL_FrMCUHWVer_enum) -> [VHAL_FrMCUHWVer_enum]
  UnitConverter138/1 -> bus_creator/150  "VHAL_FrMCUHWVer_enum"
  [VHAL_FrMCUHWVer_enum] -> UnitConverter138/1
  MCU_B_F2/10(VHAL_FrMCUSWVer_enum) -> [VHAL_FrMCUSWVer_enum]
  UnitConverter139/1 -> bus_creator/151  "VHAL_FrMCUSWVer_enum"
  [VHAL_FrMCUSWVer_enum] -> UnitConverter139/1
  MCU_B_F2/11(VHAL_FrTMTempWarn_enum) -> [VHAL_FrTMTempWarn_enum]
  UnitConverter140/1 -> bus_creator/152  "VHAL_FrTMTempWarn_enum"
  [VHAL_FrTMTempWarn_enum] -> UnitConverter140/1
  MCU_B_F2/12(VHAL_MCUBFLLCTempWarnSta_enum) -> [VHAL_MCUBFLLCTempWarnSta_enum]
  UnitConverter141/1 -> bus_creator/153  "VHAL_MCUBFLLCTempWarnSta_enum"
  [VHAL_MCUBFLLCTempWarnSta_enum] -> UnitConverter141/1
  VHAL_CANMsgInvalidMCUBR1_flg/1(Out) -> bus_creator/154
  MCU_B_R1/1(VHAL_MCUBR1CSErr_flg) -> [VHAL_MCUBR1CSErr_flg]
  UnitConverter142/1 -> bus_creator/155  "VHAL_MCUBR1CSErr_flg"
  [VHAL_MCUBR1CSErr_flg] -> UnitConverter142/1
  MCU_B_R1/2(VHAL_MCUBR1RCErr_flg) -> [VHAL_MCUBR1RCErr_flg]
  UnitConverter143/1 -> bus_creator/156  "VHAL_MCUBR1RCErr_flg"
  [VHAL_MCUBR1RCErr_flg] -> UnitConverter143/1
  MCU_B_R1/3(VHAL_MCUWarnR_enum) -> [VHAL_MCUWarnR_enum]
  UnitConverter144/1 -> bus_creator/157  "VHAL_MCUWarnR_enum"
  [VHAL_MCUWarnR_enum] -> UnitConverter144/1
  MCU_B_R1/4(VHAL_MCUBRRealPwrKwSta_kW) -> [VHAL_MCUBRRealPwrKwSta_kW]
  UnitConverter145/1 -> bus_creator/158  "VHAL_MCUBRRealPwrKwSta_kW"
  [VHAL_MCUBRRealPwrKwSta_kW] -> UnitConverter145/1
  MCU_B_R1/5(VHAL_RrActvDmpDisabSta_flg) -> [VHAL_RrActvDmpDisabSta_flg]
  UnitConverter146/1 -> bus_creator/159  "VHAL_RrActvDmpDisabSta_flg"
  [VHAL_RrActvDmpDisabSta_flg] -> UnitConverter146/1
  MCU_B_R1/6(VHAL_RrEDUDrtSta_flg) -> [VHAL_RrEDUDrtSta_flg]
  UnitConverter147/1 -> bus_creator/160  "VHAL_RrEDUDrtSta_flg"
  [VHAL_RrEDUDrtSta_flg] -> UnitConverter147/1
  MCU_B_R1/7(VHAL_RrEDUOpratingSta_flg) -> [VHAL_RrEDUOpratingSta_flg]
  UnitConverter148/1 -> bus_creator/161  "VHAL_RrEDUOpratingSta_flg"
  [VHAL_RrEDUOpratingSta_flg] -> UnitConverter148/1
  MCU_B_R1/8(VHAL_RrEDURealTMTq_Nm) -> [VHAL_RrEDURealTMTq_Nm]
  UnitConverter149/1 -> bus_creator/162  "VHAL_RrEDURealTMTq_Nm"
  [VHAL_RrEDURealTMTq_Nm] -> UnitConverter149/1
  MCU_B_R1/9(VHAL_RrEDURotateDirction_enum) -> [VHAL_RrEDURotateDirction_enum]
  UnitConverter150/1 -> bus_creator/163  "VHAL_RrEDURotateDirction_enum"
  [VHAL_RrEDURotateDirction_enum] -> UnitConverter150/1
  MCU_B_R1/10(VHAL_RrEDUTqReqFbk_Nm) -> [VHAL_RrEDUTqReqFbk_Nm]
  UnitConverter151/1 -> bus_creator/164  "VHAL_RrEDUTqReqFbk_Nm"
  [VHAL_RrEDUTqReqFbk_Nm] -> UnitConverter151/1
  MCU_B_R1/11(VHAL_RrMCU1Chksum_enum) -> [VHAL_RrMCU1Chksum_enum]
  UnitConverter152/1 -> bus_creator/165  "VHAL_RrMCU1Chksum_enum"
  [VHAL_RrMCU1Chksum_enum] -> UnitConverter152/1
  MCU_B_R1/12(VHAL_RrMCU1RolCnt_enum) -> [VHAL_RrMCU1RolCnt_enum]
  UnitConverter153/1 -> bus_creator/166  "VHAL_RrMCU1RolCnt_enum"
  [VHAL_RrMCU1RolCnt_enum] -> UnitConverter153/1
  MCU_B_R1/13(VHAL_RrMCUBAT_V) -> [VHAL_RrMCUBAT_V]
  UnitConverter154/1 -> bus_creator/167  "VHAL_RrMCUBAT_V"
  [VHAL_RrMCUBAT_V] -> UnitConverter154/1
  MCU_B_R1/14(VHAL_RrMCUDCBusCurr_A) -> [VHAL_RrMCUDCBusCurr_A]
  UnitConverter155/1 -> bus_creator/168  "VHAL_RrMCUDCBusCurr_A"
  [VHAL_RrMCUDCBusCurr_A] -> UnitConverter155/1
  MCU_B_R1/15(VHAL_RrMCUDCBusVolt_V) -> [VHAL_RrMCUDCBusVolt_V]
  UnitConverter156/1 -> bus_creator/169  "VHAL_RrMCUDCBusVolt_V"
  [VHAL_RrMCUDCBusVolt_V] -> UnitConverter156/1
  MCU_B_R1/16(VHAL_RrMCUDischrgSta_flg) -> [VHAL_RrMCUDischrgSta_flg]
  UnitConverter157/1 -> bus_creator/170  "VHAL_RrMCUDischrgSta_flg"
  [VHAL_RrMCUDischrgSta_flg] -> UnitConverter157/1
  MCU_B_R1/17(VHAL_RrMCUEnaSta_flg) -> [VHAL_RrMCUEnaSta_flg]
  UnitConverter158/1 -> bus_creator/171  "VHAL_RrMCUEnaSta_flg"
  [VHAL_RrMCUEnaSta_flg] -> UnitConverter158/1
  MCU_B_R1/18(VHAL_RrMCUErr_enum) -> [VHAL_RrMCUErr_enum]
  UnitConverter159/1 -> bus_creator/172  "VHAL_RrMCUErr_enum"
  [VHAL_RrMCUErr_enum] -> UnitConverter159/1
  MCU_B_R1/19(VHAL_RrMCUIGNsta_flg) -> [VHAL_RrMCUIGNsta_flg]
  UnitConverter160/1 -> bus_creator/173  "VHAL_RrMCUIGNsta_flg"
  [VHAL_RrMCUIGNsta_flg] -> UnitConverter160/1
  MCU_B_R1/20(VHAL_RrMCUReady_flg) -> [VHAL_RrMCUReady_flg]
  UnitConverter161/1 -> bus_creator/174  "VHAL_RrMCUReady_flg"
  [VHAL_RrMCUReady_flg] -> UnitConverter161/1
  MCU_B_R1/21(VHAL_RrMCUReady4Pre_flg) -> [VHAL_RrMCUReady4Pre_flg]
  UnitConverter162/1 -> bus_creator/175  "VHAL_RrMCUReady4Pre_flg"
  [VHAL_RrMCUReady4Pre_flg] -> UnitConverter162/1
  MCU_B_R1/22(VHAL_RrMCUSysSta_enum) -> [VHAL_RrMCUSysSta_enum]
  UnitConverter163/1 -> bus_creator/176  "VHAL_RrMCUSysSta_enum"
  [VHAL_RrMCUSysSta_enum] -> UnitConverter163/1
  MCU_B_R1/23(VHAL_RrMCUTemp_C) -> [VHAL_RrMCUTemp_C]
  UnitConverter164/1 -> bus_creator/177  "VHAL_RrMCUTemp_C"
  [VHAL_RrMCUTemp_C] -> UnitConverter164/1
  MCU_B_R1/24(VHAL_RrMotorAvailTq_Nm) -> [VHAL_RrMotorAvailTq_Nm]
  UnitConverter165/1 -> bus_creator/178  "VHAL_RrMotorAvailTq_Nm"
  [VHAL_RrMotorAvailTq_Nm] -> UnitConverter165/1
  MCU_B_R1/25(VHAL_RrRegenAvailTq_Nm) -> [VHAL_RrRegenAvailTq_Nm]
  UnitConverter166/1 -> bus_creator/179  "VHAL_RrRegenAvailTq_Nm"
  [VHAL_RrRegenAvailTq_Nm] -> UnitConverter166/1
  MCU_B_R1/26(VHAL_RrTMSpd_rpm) -> [VHAL_RrTMSpd_rpm]
  UnitConverter167/1 -> bus_creator/180  "VHAL_RrTMSpd_rpm"
  [VHAL_RrTMSpd_rpm] -> UnitConverter167/1
  MCU_B_R1/27(VHAL_RrTMTemp_C) -> [VHAL_RrTMTemp_C]
  UnitConverter168/1 -> bus_creator/181  "VHAL_RrTMTemp_C"
  [VHAL_RrTMTemp_C] -> UnitConverter168/1
  MCU_B_R1/28(VHAL_RrTMid_A) -> [VHAL_RrTMid_A]
  UnitConverter169/1 -> bus_creator/182  "VHAL_RrTMid_A"
  [VHAL_RrTMid_A] -> UnitConverter169/1
  MCU_B_R1/29(VHAL_RrTMiq_A) -> [VHAL_RrTMiq_A]
  UnitConverter170/1 -> bus_creator/183  "VHAL_RrTMiq_A"
  [VHAL_RrTMiq_A] -> UnitConverter170/1
  VHAL_CANMsgInvalidMCUBR2_flg/1(Out) -> bus_creator/184
  MCU_B_R2/1(VHAL_MCUBRLLCTempWarnSta_enum) -> [VHAL_MCUBRLLCTempWarnSta_enum]
  UnitConverter171/1 -> bus_creator/185  "VHAL_MCUBRLLCTempWarnSta_enum"
  [VHAL_MCUBRLLCTempWarnSta_enum] -> UnitConverter171/1
  MCU_B_R2/2(VHAL_RrCoolanttempReq_cnt) -> [VHAL_RrCoolanttempReq_cnt]
  UnitConverter172/1 -> bus_creator/186  "VHAL_RrCoolanttempReq_cnt"
  [VHAL_RrCoolanttempReq_cnt] -> UnitConverter172/1
  MCU_B_R2/3(VHAL_RrFailcode1_enum) -> [VHAL_RrFailcode1_enum]
  UnitConverter173/1 -> bus_creator/187  "VHAL_RrFailcode1_enum"
  [VHAL_RrFailcode1_enum] -> UnitConverter173/1
  MCU_B_R2/4(VHAL_RrFailcode2_enum) -> [VHAL_RrFailcode2_enum]
  UnitConverter174/1 -> bus_creator/188  "VHAL_RrFailcode2_enum"
  [VHAL_RrFailcode2_enum] -> UnitConverter174/1
  MCU_B_R2/5(VHAL_RrFailcodehistory1_enum) -> [VHAL_RrFailcodehistory1_enum]
  UnitConverter175/1 -> bus_creator/189  "VHAL_RrFailcodehistory1_enum"
  [VHAL_RrFailcodehistory1_enum] -> UnitConverter175/1
  MCU_B_R2/6(VHAL_RrFailcodehistory2_enum) -> [VHAL_RrFailcodehistory2_enum]
  UnitConverter176/1 -> bus_creator/190  "VHAL_RrFailcodehistory2_enum"
  [VHAL_RrFailcodehistory2_enum] -> UnitConverter176/1
  MCU_B_R2/7(VHAL_RrLLCTemp_C) -> [VHAL_RrLLCTemp_C]
  UnitConverter177/1 -> bus_creator/191  "VHAL_RrLLCTemp_C"
  [VHAL_RrLLCTemp_C] -> UnitConverter177/1
  MCU_B_R2/8(VHAL_RrLLCflowReq_Lpmin) -> [VHAL_RrLLCflowReq_Lpmin]
  UnitConverter178/1 -> bus_creator/192  "VHAL_RrLLCflowReq_Lpmin"
  [VHAL_RrLLCflowReq_Lpmin] -> UnitConverter178/1
  MCU_B_R2/9(VHAL_RrMCU3HWVer_enum) -> [VHAL_RrMCU3HWVer_enum]
  UnitConverter179/1 -> bus_creator/193  "VHAL_RrMCU3HWVer_enum"
  [VHAL_RrMCU3HWVer_enum] -> UnitConverter179/1
  MCU_B_R2/10(VHAL_RrMCU3SWVer_enum) -> [VHAL_RrMCU3SWVer_enum]
  UnitConverter180/1 -> bus_creator/194  "VHAL_RrMCU3SWVer_enum"
  [VHAL_RrMCU3SWVer_enum] -> UnitConverter180/1
  MCU_B_R2/11(VHAL_RrMCUTempWarn_enum) -> [VHAL_RrMCUTempWarn_enum]
  UnitConverter181/1 -> bus_creator/195  "VHAL_RrMCUTempWarn_enum"
  [VHAL_RrMCUTempWarn_enum] -> UnitConverter181/1
  MCU_B_R2/12(VHAL_RrTMTempWarn_enum) -> [VHAL_RrTMTempWarn_enum]
  UnitConverter182/1 -> bus_creator/196  "VHAL_RrTMTempWarn_enum"
  [VHAL_RrTMTempWarn_enum] -> UnitConverter182/1
  VHAL_CANMsgInvalidMCUNF1_flg/1(Out) -> bus_creator/197
  MCU_N_F1/1(VHAL_MCUNF1CSErr_flg) -> [VHAL_MCUNF1CSErr_flg]
  UnitConverter183/1 -> bus_creator/198  "VHAL_MCUNF1CSErr_flg"
  [VHAL_MCUNF1CSErr_flg] -> UnitConverter183/1
  MCU_N_F1/2(VHAL_MCUNF1RCErr_flg) -> [VHAL_MCUNF1RCErr_flg]
  UnitConverter184/1 -> bus_creator/199  "VHAL_MCUNF1RCErr_flg"
  [VHAL_MCUNF1RCErr_flg] -> UnitConverter184/1
  MCU_N_F1/3(VHAL_FrActvDmpDisabStaNidec_flg) -> [VHAL_FrActvDmpDisabStaNidec_flg]
  UnitConverter185/1 -> bus_creator/200  "VHAL_FrActvDmpDisabStaNidec_flg"
  [VHAL_FrActvDmpDisabStaNidec_flg] -> UnitConverter185/1
  MCU_N_F1/4(VHAL_FrEDUDrtStaNidec_flg) -> [VHAL_FrEDUDrtStaNidec_flg]
  UnitConverter186/1 -> bus_creator/201  "VHAL_FrEDUDrtStaNidec_flg"
  [VHAL_FrEDUDrtStaNidec_flg] -> UnitConverter186/1
  MCU_N_F1/5(VHAL_FrEDUOpratingStaNidec_flg) -> [VHAL_FrEDUOpratingStaNidec_flg]
  UnitConverter187/1 -> bus_creator/202  "VHAL_FrEDUOpratingStaNidec_flg"
  [VHAL_FrEDUOpratingStaNidec_flg] -> UnitConverter187/1
  MCU_N_F1/6(VHAL_FrEDURealTMTqNidec_Nm) -> [VHAL_FrEDURealTMTqNidec_Nm]
  UnitConverter188/1 -> bus_creator/203  "VHAL_FrEDURealTMTqNidec_Nm"
  [VHAL_FrEDURealTMTqNidec_Nm] -> UnitConverter188/1
  MCU_N_F1/7(VHAL_FrEDURotateDirctionNidec_enum) -> [VHAL_FrEDURotateDirctionNidec_enum]
  UnitConverter189/1 -> bus_creator/204  "VHAL_FrEDURotateDirctionNidec_enum"
  [VHAL_FrEDURotateDirctionNidec_enum] -> UnitConverter189/1
  MCU_N_F1/8(VHAL_FrEDUTqReqFbkNidec_Nm) -> [VHAL_FrEDUTqReqFbkNidec_Nm]
  UnitConverter190/1 -> bus_creator/205  "VHAL_FrEDUTqReqFbkNidec_Nm"
  [VHAL_FrEDUTqReqFbkNidec_Nm] -> UnitConverter190/1
  MCU_N_F1/9(VHAL_FrMCU1ChksumNidec_enum) -> [VHAL_FrMCU1ChksumNidec_enum]
  UnitConverter191/1 -> bus_creator/206  "VHAL_FrMCU1ChksumNidec_enum"
  [VHAL_FrMCU1ChksumNidec_enum] -> UnitConverter191/1
  MCU_N_F1/10(VHAL_FrMCU1RolCntNidec_enum) -> [VHAL_FrMCU1RolCntNidec_enum]
  UnitConverter192/1 -> bus_creator/207  "VHAL_FrMCU1RolCntNidec_enum"
  [VHAL_FrMCU1RolCntNidec_enum] -> UnitConverter192/1
  MCU_N_F1/11(VHAL_FrMCUBATNidec_V) -> [VHAL_FrMCUBATNidec_V]
  UnitConverter193/1 -> bus_creator/208  "VHAL_FrMCUBATNidec_V"
  [VHAL_FrMCUBATNidec_V] -> UnitConverter193/1
  MCU_N_F1/12(VHAL_FrMCUDCBusCurrNidec_A) -> [VHAL_FrMCUDCBusCurrNidec_A]
  UnitConverter194/1 -> bus_creator/209  "VHAL_FrMCUDCBusCurrNidec_A"
  [VHAL_FrMCUDCBusCurrNidec_A] -> UnitConverter194/1
  MCU_N_F1/13(VHAL_FrMCUDCBusVoltNidec_V) -> [VHAL_FrMCUDCBusVoltNidec_V]
  UnitConverter195/1 -> bus_creator/210  "VHAL_FrMCUDCBusVoltNidec_V"
  [VHAL_FrMCUDCBusVoltNidec_V] -> UnitConverter195/1
  MCU_N_F1/14(VHAL_FrMCUDischrgStaNidec_flg) -> [VHAL_FrMCUDischrgStaNidec_flg]
  UnitConverter196/1 -> bus_creator/211  "VHAL_FrMCUDischrgStaNidec_flg"
  [VHAL_FrMCUDischrgStaNidec_flg] -> UnitConverter196/1
  MCU_N_F1/15(VHAL_FrMCUEnaStaNidec_flg) -> [VHAL_FrMCUEnaStaNidec_flg]
  UnitConverter197/1 -> bus_creator/212  "VHAL_FrMCUEnaStaNidec_flg"
  [VHAL_FrMCUEnaStaNidec_flg] -> UnitConverter197/1
  MCU_N_F1/16(VHAL_FrMCUErrNidec_enum) -> [VHAL_FrMCUErrNidec_enum]
  UnitConverter198/1 -> bus_creator/213  "VHAL_FrMCUErrNidec_enum"
  [VHAL_FrMCUErrNidec_enum] -> UnitConverter198/1
  MCU_N_F1/17(VHAL_FrMCUIGNstaNidec_flg) -> [VHAL_FrMCUIGNstaNidec_flg]
  UnitConverter199/1 -> bus_creator/214  "VHAL_FrMCUIGNstaNidec_flg"
  [VHAL_FrMCUIGNstaNidec_flg] -> UnitConverter199/1
  MCU_N_F1/18(VHAL_FrMCUReady4PreNidec_flg) -> [VHAL_FrMCUReady4PreNidec_flg]
  UnitConverter200/1 -> bus_creator/215  "VHAL_FrMCUReady4PreNidec_flg"
  [VHAL_FrMCUReady4PreNidec_flg] -> UnitConverter200/1
  MCU_N_F1/19(VHAL_FrMCUReadyNidec_flg) -> [VHAL_FrMCUReadyNidec_flg]
  UnitConverter201/1 -> bus_creator/216  "VHAL_FrMCUReadyNidec_flg"
  [VHAL_FrMCUReadyNidec_flg] -> UnitConverter201/1
  MCU_N_F1/20(VHAL_FrMCUSysStaNidec_enum) -> [VHAL_FrMCUSysStaNidec_enum]
  UnitConverter202/1 -> bus_creator/217  "VHAL_FrMCUSysStaNidec_enum"
  [VHAL_FrMCUSysStaNidec_enum] -> UnitConverter202/1
  MCU_N_F1/21(VHAL_FrMCUTempNidec_C) -> [VHAL_FrMCUTempNidec_C]
  UnitConverter203/1 -> bus_creator/218  "VHAL_FrMCUTempNidec_C"
  [VHAL_FrMCUTempNidec_C] -> UnitConverter203/1
  MCU_N_F1/22(VHAL_FrMotorAvailTqNidec_Nm) -> [VHAL_FrMotorAvailTqNidec_Nm]
  UnitConverter204/1 -> bus_creator/219  "VHAL_FrMotorAvailTqNidec_Nm"
  [VHAL_FrMotorAvailTqNidec_Nm] -> UnitConverter204/1
  MCU_N_F1/23(VHAL_FrRegenAvailTqNidec_Nm) -> [VHAL_FrRegenAvailTqNidec_Nm]
  UnitConverter205/1 -> bus_creator/220  "VHAL_FrRegenAvailTqNidec_Nm"
  [VHAL_FrRegenAvailTqNidec_Nm] -> UnitConverter205/1
  MCU_N_F1/24(VHAL_FrTMSpdNidec_rpm) -> [VHAL_FrTMSpdNidec_rpm]
  UnitConverter206/1 -> bus_creator/221  "VHAL_FrTMSpdNidec_rpm"
  [VHAL_FrTMSpdNidec_rpm] -> UnitConverter206/1
  MCU_N_F1/25(VHAL_FrTMTempNidec_C) -> [VHAL_FrTMTempNidec_C]
  UnitConverter207/1 -> bus_creator/222  "VHAL_FrTMTempNidec_C"
  [VHAL_FrTMTempNidec_C] -> UnitConverter207/1
  MCU_N_F1/26(VHAL_FrTMidNidec_A) -> [VHAL_FrTMidNidec_A]
  UnitConverter208/1 -> bus_creator/223  "VHAL_FrTMidNidec_A"
  [VHAL_FrTMidNidec_A] -> UnitConverter208/1
  MCU_N_F1/27(VHAL_FrTMiqNidec_A) -> [VHAL_FrTMiqNidec_A]
  UnitConverter209/1 -> bus_creator/224  "VHAL_FrTMiqNidec_A"
  [VHAL_FrTMiqNidec_A] -> UnitConverter209/1
  MCU_N_F1/28(VHAL_MCUWarnFNidec_enum) -> [VHAL_MCUWarnFNidec_enum]
  UnitConverter210/1 -> bus_creator/225  "VHAL_MCUWarnFNidec_enum"
  [VHAL_MCUWarnFNidec_enum] -> UnitConverter210/1
  VHAL_CANMsgInvalidMCUNF2_flg/1(Out) -> bus_creator/226
  MCU_N_F2/1(VHAL_FrCoolanttempReqNidec_C) -> [VHAL_FrCoolanttempReqNidec_C]
  UnitConverter211/1 -> bus_creator/227  "VHAL_FrCoolanttempReqNidec_C"
  [VHAL_FrCoolanttempReqNidec_C] -> UnitConverter211/1
  MCU_N_F2/2(VHAL_FrEOPSpdSetNidec_rpm) -> [VHAL_FrEOPSpdSetNidec_rpm]
  UnitConverter212/1 -> bus_creator/228  "VHAL_FrEOPSpdSetNidec_rpm"
  [VHAL_FrEOPSpdSetNidec_rpm] -> UnitConverter212/1
  MCU_N_F2/3(VHAL_FrFailcode1Nidec_enum) -> [VHAL_FrFailcode1Nidec_enum]
  UnitConverter213/1 -> bus_creator/229  "VHAL_FrFailcode1Nidec_enum"
  [VHAL_FrFailcode1Nidec_enum] -> UnitConverter213/1
  MCU_N_F2/4(VHAL_FrFailcode2Nidec_enum) -> [VHAL_FrFailcode2Nidec_enum]
  UnitConverter214/1 -> bus_creator/230  "VHAL_FrFailcode2Nidec_enum"
  [VHAL_FrFailcode2Nidec_enum] -> UnitConverter214/1
  MCU_N_F2/5(VHAL_FrFailcodehistory1Nidec_enum) -> [VHAL_FrFailcodehistory1Nidec_enum]
  UnitConverter215/1 -> bus_creator/231  "VHAL_FrFailcodehistory1Nidec_enum"
  [VHAL_FrFailcodehistory1Nidec_enum] -> UnitConverter215/1
  MCU_N_F2/6(VHAL_FrFailcodehistory2Nidec_enum) -> [VHAL_FrFailcodehistory2Nidec_enum]
  UnitConverter216/1 -> bus_creator/232  "VHAL_FrFailcodehistory2Nidec_enum"
  [VHAL_FrFailcodehistory2Nidec_enum] -> UnitConverter216/1
  MCU_N_F2/7(VHAL_FrLLCTempNidec_C) -> [VHAL_FrLLCTempNidec_C]
  UnitConverter217/1 -> bus_creator/233  "VHAL_FrLLCTempNidec_C"
  [VHAL_FrLLCTempNidec_C] -> UnitConverter217/1
  MCU_N_F2/8(VHAL_FrLLCflowReqNidec_Lpmin) -> [VHAL_FrLLCflowReqNidec_Lpmin]
  UnitConverter218/1 -> bus_creator/234  "VHAL_FrLLCflowReqNidec_Lpmin"
  [VHAL_FrLLCflowReqNidec_Lpmin] -> UnitConverter218/1
  MCU_N_F2/9(VHAL_FrMCUTempWarnNidec_enum) -> [VHAL_FrMCUTempWarnNidec_enum]
  UnitConverter219/1 -> bus_creator/235  "VHAL_FrMCUTempWarnNidec_enum"
  [VHAL_FrMCUTempWarnNidec_enum] -> UnitConverter219/1
  MCU_N_F2/10(VHAL_FrTMTempWarnNidec_enum) -> [VHAL_FrTMTempWarnNidec_enum]
  UnitConverter220/1 -> bus_creator/236  "VHAL_FrTMTempWarnNidec_enum"
  [VHAL_FrTMTempWarnNidec_enum] -> UnitConverter220/1
  VHAL_CANMsgInvalidMCUNF3_flg/1(Out) -> bus_creator/237
  MCU_N_F3/1(VHAL_FrMCUHWVerNidec_enum) -> [VHAL_FrMCUHWVerNidec_enum]
  UnitConverter221/1 -> bus_creator/238  "VHAL_FrMCUHWVerNidec_enum"
  [VHAL_FrMCUHWVerNidec_enum] -> UnitConverter221/1
  MCU_N_F3/2(VHAL_FrMCUSWVerNidec_enum) -> [VHAL_FrMCUSWVerNidec_enum]
  UnitConverter222/1 -> bus_creator/239  "VHAL_FrMCUSWVerNidec_enum"
  [VHAL_FrMCUSWVerNidec_enum] -> UnitConverter222/1
  VHAL_CANMsgInvalidMCUNR1_flg/1(Out) -> bus_creator/240
  MCU_N_R1/1(VHAL_MCUNR1CSErr_flg) -> [VHAL_MCUNR1CSErr_flg]
  UnitConverter223/1 -> bus_creator/241  "VHAL_MCUNR1CSErr_flg"
  [VHAL_MCUNR1CSErr_flg] -> UnitConverter223/1
  MCU_N_R1/2(VHAL_MCUNR1RCErr_flg) -> [VHAL_MCUNR1RCErr_flg]
  UnitConverter224/1 -> bus_creator/242  "VHAL_MCUNR1RCErr_flg"
  [VHAL_MCUNR1RCErr_flg] -> UnitConverter224/1
  MCU_N_R1/3(VHAL_MCUWarnRNidec_enum) -> [VHAL_MCUWarnRNidec_enum]
  UnitConverter225/1 -> bus_creator/243  "VHAL_MCUWarnRNidec_enum"
  [VHAL_MCUWarnRNidec_enum] -> UnitConverter225/1
  MCU_N_R1/4(VHAL_RrActvDmpDisabStaNidec_flg) -> [VHAL_RrActvDmpDisabStaNidec_flg]
  UnitConverter226/1 -> bus_creator/244  "VHAL_RrActvDmpDisabStaNidec_flg"
  [VHAL_RrActvDmpDisabStaNidec_flg] -> UnitConverter226/1
  MCU_N_R1/5(VHAL_RrEDUDrtStaNidec_flg) -> [VHAL_RrEDUDrtStaNidec_flg]
  UnitConverter227/1 -> bus_creator/245  "VHAL_RrEDUDrtStaNidec_flg"
  [VHAL_RrEDUDrtStaNidec_flg] -> UnitConverter227/1
  MCU_N_R1/6(VHAL_RrEDUOpratingStaNidec_flg) -> [VHAL_RrEDUOpratingStaNidec_flg]
  UnitConverter228/1 -> bus_creator/246  "VHAL_RrEDUOpratingStaNidec_flg"
  [VHAL_RrEDUOpratingStaNidec_flg] -> UnitConverter228/1
  MCU_N_R1/7(VHAL_RrEDURealTMTqNidec_Nm) -> [VHAL_RrEDURealTMTqNidec_Nm]
  UnitConverter229/1 -> bus_creator/247  "VHAL_RrEDURealTMTqNidec_Nm"
  [VHAL_RrEDURealTMTqNidec_Nm] -> UnitConverter229/1
  MCU_N_R1/8(VHAL_RrEDURotateDirctionNidec_enum) -> [VHAL_RrEDURotateDirctionNidec_enum]
  UnitConverter230/1 -> bus_creator/248  "VHAL_RrEDURotateDirctionNidec_enum"
  [VHAL_RrEDURotateDirctionNidec_enum] -> UnitConverter230/1
  MCU_N_R1/9(VHAL_RrEDUTqReqFbkNidec_Nm) -> [VHAL_RrEDUTqReqFbkNidec_Nm]
  UnitConverter231/1 -> bus_creator/249  "VHAL_RrEDUTqReqFbkNidec_Nm"
  [VHAL_RrEDUTqReqFbkNidec_Nm] -> UnitConverter231/1
  MCU_N_R1/10(VHAL_RrMCU1ChksumNidec_enum) -> [VHAL_RrMCU1ChksumNidec_enum]
  UnitConverter232/1 -> bus_creator/250  "VHAL_RrMCU1ChksumNidec_enum"
  [VHAL_RrMCU1ChksumNidec_enum] -> UnitConverter232/1
  MCU_N_R1/11(VHAL_RrMCU1RolCntNidec_enum) -> [VHAL_RrMCU1RolCntNidec_enum]
  UnitConverter233/1 -> bus_creator/251  "VHAL_RrMCU1RolCntNidec_enum"
  [VHAL_RrMCU1RolCntNidec_enum] -> UnitConverter233/1
  MCU_N_R1/12(VHAL_RrMCUBATNidec_V) -> [VHAL_RrMCUBATNidec_V]
  UnitConverter234/1 -> bus_creator/252  "VHAL_RrMCUBATNidec_V"
  [VHAL_RrMCUBATNidec_V] -> UnitConverter234/1
  MCU_N_R1/13(VHAL_RrMCUDCBusCurrNidec_A) -> [VHAL_RrMCUDCBusCurrNidec_A]
  UnitConverter235/1 -> bus_creator/253  "VHAL_RrMCUDCBusCurrNidec_A"
  [VHAL_RrMCUDCBusCurrNidec_A] -> UnitConverter235/1
  MCU_N_R1/14(VHAL_RrMCUDCBusVoltNidec_V) -> [VHAL_RrMCUDCBusVoltNidec_V]
  UnitConverter236/1 -> bus_creator/254  "VHAL_RrMCUDCBusVoltNidec_V"
  [VHAL_RrMCUDCBusVoltNidec_V] -> UnitConverter236/1
  MCU_N_R1/15(VHAL_RrMCUDischrgStaNidec_flg) -> [VHAL_RrMCUDischrgStaNidec_flg]
  UnitConverter237/1 -> bus_creator/255  "VHAL_RrMCUDischrgStaNidec_flg"
  [VHAL_RrMCUDischrgStaNidec_flg] -> UnitConverter237/1
  MCU_N_R1/16(VHAL_RrMCUEnaStaNidec_flg) -> [VHAL_RrMCUEnaStaNidec_flg]
  UnitConverter238/1 -> bus_creator/256  "VHAL_RrMCUEnaStaNidec_flg"
  [VHAL_RrMCUEnaStaNidec_flg] -> UnitConverter238/1
  MCU_N_R1/17(VHAL_RrMCUErrNidec_enum) -> [VHAL_RrMCUErrNidec_enum]
  UnitConverter239/1 -> bus_creator/257  "VHAL_RrMCUErrNidec_enum"
  [VHAL_RrMCUErrNidec_enum] -> UnitConverter239/1
  MCU_N_R1/18(VHAL_RrMCUIGNstaNidec_flg) -> [VHAL_RrMCUIGNstaNidec_flg]
  UnitConverter240/1 -> bus_creator/258  "VHAL_RrMCUIGNstaNidec_flg"
  [VHAL_RrMCUIGNstaNidec_flg] -> UnitConverter240/1
  MCU_N_R1/19(VHAL_RrMCUReady4PreNidec_flg) -> [VHAL_RrMCUReady4PreNidec_flg]
  UnitConverter241/1 -> bus_creator/259  "VHAL_RrMCUReady4PreNidec_flg"
  [VHAL_RrMCUReady4PreNidec_flg] -> UnitConverter241/1
  MCU_N_R1/20(VHAL_RrMCUReadyNidec_flg) -> [VHAL_RrMCUReadyNidec_flg]
  UnitConverter242/1 -> bus_creator/260  "VHAL_RrMCUReadyNidec_flg"
  [VHAL_RrMCUReadyNidec_flg] -> UnitConverter242/1
  MCU_N_R1/21(VHAL_RrMCUSysStaNidec_enum) -> [VHAL_RrMCUSysStaNidec_enum]
  UnitConverter243/1 -> bus_creator/261  "VHAL_RrMCUSysStaNidec_enum"
  [VHAL_RrMCUSysStaNidec_enum] -> UnitConverter243/1
  MCU_N_R1/22(VHAL_RrMCUTempNidec_C) -> [VHAL_RrMCUTempNidec_C]
  UnitConverter244/1 -> bus_creator/262  "VHAL_RrMCUTempNidec_C"
  [VHAL_RrMCUTempNidec_C] -> UnitConverter244/1
  MCU_N_R1/23(VHAL_RrMotorAvailTqNidec_Nm) -> [VHAL_RrMotorAvailTqNidec_Nm]
  UnitConverter245/1 -> bus_creator/263  "VHAL_RrMotorAvailTqNidec_Nm"
  [VHAL_RrMotorAvailTqNidec_Nm] -> UnitConverter245/1
  MCU_N_R1/24(VHAL_RrRegenAvailTqNidec_Nm) -> [VHAL_RrRegenAvailTqNidec_Nm]
  UnitConverter246/1 -> bus_creator/264  "VHAL_RrRegenAvailTqNidec_Nm"
  [VHAL_RrRegenAvailTqNidec_Nm] -> UnitConverter246/1
  MCU_N_R1/25(VHAL_RrTMSpdNidec_rpm) -> [VHAL_RrTMSpdNidec_rpm]
  UnitConverter247/1 -> bus_creator/265  "VHAL_RrTMSpdNidec_rpm"
  [VHAL_RrTMSpdNidec_rpm] -> UnitConverter247/1
  MCU_N_R1/26(VHAL_RrTMTempNidec_C) -> [VHAL_RrTMTempNidec_C]
  UnitConverter248/1 -> bus_creator/266  "VHAL_RrTMTempNidec_C"
  [VHAL_RrTMTempNidec_C] -> UnitConverter248/1
  MCU_N_R1/27(VHAL_RrTMidNidec_A) -> [VHAL_RrTMidNidec_A]
  UnitConverter249/1 -> bus_creator/267  "VHAL_RrTMidNidec_A"
  [VHAL_RrTMidNidec_A] -> UnitConverter249/1
  MCU_N_R1/28(VHAL_RrTMiqNidec_A) -> [VHAL_RrTMiqNidec_A]
  UnitConverter250/1 -> bus_creator/268  "VHAL_RrTMiqNidec_A"
  [VHAL_RrTMiqNidec_A] -> UnitConverter250/1
  VHAL_CANMsgInvalidMCUNR2_flg/1(Out) -> bus_creator/269
  MCU_N_R2/1(VHAL_RrCoolanttempReqNidec_cnt) -> [VHAL_RrCoolanttempReqNidec_cnt]
  UnitConverter251/1 -> bus_creator/270  "VHAL_RrCoolanttempReqNidec_cnt"
  [VHAL_RrCoolanttempReqNidec_cnt] -> UnitConverter251/1
  MCU_N_R2/2(VHAL_RrEOPSpdSetNidec_rpm) -> [VHAL_RrEOPSpdSetNidec_rpm]
  UnitConverter252/1 -> bus_creator/271  "VHAL_RrEOPSpdSetNidec_rpm"
  [VHAL_RrEOPSpdSetNidec_rpm] -> UnitConverter252/1
  MCU_N_R2/3(VHAL_RrFailcode1Nidec_enum) -> [VHAL_RrFailcode1Nidec_enum]
  UnitConverter253/1 -> bus_creator/272  "VHAL_RrFailcode1Nidec_enum"
  [VHAL_RrFailcode1Nidec_enum] -> UnitConverter253/1
  MCU_N_R2/4(VHAL_RrFailcode2Nidec_enum) -> [VHAL_RrFailcode2Nidec_enum]
  UnitConverter254/1 -> bus_creator/273  "VHAL_RrFailcode2Nidec_enum"
  [VHAL_RrFailcode2Nidec_enum] -> UnitConverter254/1
  MCU_N_R2/5(VHAL_RrFailcodehistory1Nidec_enum) -> [VHAL_RrFailcodehistory1Nidec_enum]
  UnitConverter255/1 -> bus_creator/274  "VHAL_RrFailcodehistory1Nidec_enum"
  [VHAL_RrFailcodehistory1Nidec_enum] -> UnitConverter255/1
  MCU_N_R2/6(VHAL_RrFailcodehistory2Nidec_enum) -> [VHAL_RrFailcodehistory2Nidec_enum]
  UnitConverter256/1 -> bus_creator/275  "VHAL_RrFailcodehistory2Nidec_enum"
  [VHAL_RrFailcodehistory2Nidec_enum] -> UnitConverter256/1
  MCU_N_R2/7(VHAL_RrLLCTempNidec_C) -> [VHAL_RrLLCTempNidec_C]
  UnitConverter257/1 -> bus_creator/276  "VHAL_RrLLCTempNidec_C"
  [VHAL_RrLLCTempNidec_C] -> UnitConverter257/1
  MCU_N_R2/8(VHAL_RrLLCflowReqNidec_Lpmin) -> [VHAL_RrLLCflowReqNidec_Lpmin]
  UnitConverter258/1 -> bus_creator/277  "VHAL_RrLLCflowReqNidec_Lpmin"
  [VHAL_RrLLCflowReqNidec_Lpmin] -> UnitConverter258/1
  MCU_N_R2/9(VHAL_RrMCUTempWarnNidec_enum) -> [VHAL_RrMCUTempWarnNidec_enum]
  UnitConverter259/1 -> bus_creator/278  "VHAL_RrMCUTempWarnNidec_enum"
  [VHAL_RrMCUTempWarnNidec_enum] -> UnitConverter259/1
  MCU_N_R2/10(VHAL_RrTMTempWarnNidec_enum) -> [VHAL_RrTMTempWarnNidec_enum]
  UnitConverter260/1 -> bus_creator/279  "VHAL_RrTMTempWarnNidec_enum"
  [VHAL_RrTMTempWarnNidec_enum] -> UnitConverter260/1
  VHAL_CANMsgInvalidMCUNR3_flg/1(Out) -> bus_creator/280
  MCU_N_R3/1(VHAL_RrMCU3HWVerNidec_enum) -> [VHAL_RrMCU3HWVerNidec_enum]
  UnitConverter261/1 -> bus_creator/281  "VHAL_RrMCU3HWVerNidec_enum"
  [VHAL_RrMCU3HWVerNidec_enum] -> UnitConverter261/1
  MCU_N_R3/2(VHAL_RrMCU3SWVerNidec_enum) -> [VHAL_RrMCU3SWVerNidec_enum]
  UnitConverter262/1 -> bus_creator/282  "VHAL_RrMCU3SWVerNidec_enum"
  [VHAL_RrMCU3SWVerNidec_enum] -> UnitConverter262/1
  VHAL_CANMsgInvalidShifter1_flg/1(Out) -> bus_creator/283
  Shifter1/1(VHAL_Shifter1CSErr_flg) -> [VHAL_Shifter1CSErr_flg]
  UnitConverter263/1 -> bus_creator/284  "VHAL_Shifter1CSErr_flg"
  [VHAL_Shifter1CSErr_flg] -> UnitConverter263/1
  Shifter1/2(VHAL_Shifter1RCErr_flg) -> [VHAL_Shifter1RCErr_flg]
  UnitConverter264/1 -> bus_creator/285  "VHAL_Shifter1RCErr_flg"
  [VHAL_Shifter1RCErr_flg] -> UnitConverter264/1
  Shifter1/3(VHAL_ShifterCRC8_enum) -> [VHAL_ShifterCRC8_enum]
  UnitConverter265/1 -> bus_creator/286  "VHAL_ShifterCRC8_enum"
  [VHAL_ShifterCRC8_enum] -> UnitConverter265/1
  Shifter1/4(VHAL_ShifterFailsta_enum) -> [VHAL_ShifterFailsta_enum]
  UnitConverter266/1 -> bus_creator/287  "VHAL_ShifterFailsta_enum"
  [VHAL_ShifterFailsta_enum] -> UnitConverter266/1
  Shifter1/5(VHAL_ShifterHandleCmd_enum) -> [VHAL_ShifterHandleCmd_enum]
  UnitConverter267/1 -> bus_creator/288  "VHAL_ShifterHandleCmd_enum"
  [VHAL_ShifterHandleCmd_enum] -> UnitConverter267/1
  Shifter1/6(VHAL_ShifterRC_enum) -> [VHAL_ShifterRC_enum]
  UnitConverter268/1 -> bus_creator/289  "VHAL_ShifterRC_enum"
  [VHAL_ShifterRC_enum] -> UnitConverter268/1
  VHAL_CANMsgInvalidShifter2_flg/1(Out) -> bus_creator/290
  Shifter2/1(VHAL_Shifter2CSErr_flg) -> [VHAL_Shifter2CSErr_flg]
  UnitConverter269/1 -> bus_creator/291  "VHAL_Shifter2CSErr_flg"
  [VHAL_Shifter2CSErr_flg] -> UnitConverter269/1
  Shifter2/2(VHAL_Shifter2RCErr_flg) -> [VHAL_Shifter2RCErr_flg]
  UnitConverter270/1 -> bus_creator/292  "VHAL_Shifter2RCErr_flg"
  [VHAL_Shifter2RCErr_flg] -> UnitConverter270/1
  Shifter2/3(VHAL_CSW2DimSwSta_flg) -> [VHAL_CSW2DimSwSta_flg]
  UnitConverter271/1 -> bus_creator/293  "VHAL_CSW2DimSwSta_flg"
  [VHAL_CSW2DimSwSta_flg] -> UnitConverter271/1
  Shifter2/4(VHAL_CSW2FWasSwSta_enum) -> [VHAL_CSW2FWasSwSta_enum]
  UnitConverter272/1 -> bus_creator/294  "VHAL_CSW2FWasSwSta_enum"
  [VHAL_CSW2FWasSwSta_enum] -> UnitConverter272/1
  Shifter2/5(VHAL_CSW2FWipSwSta_enum) -> [VHAL_CSW2FWipSwSta_enum]
  UnitConverter273/1 -> bus_creator/295  "VHAL_CSW2FWipSwSta_enum"
  [VHAL_CSW2FWipSwSta_enum] -> UnitConverter273/1
  Shifter2/6(VHAL_CSW2PassSWSta_flg) -> [VHAL_CSW2PassSWSta_flg]
  UnitConverter274/1 -> bus_creator/296  "VHAL_CSW2PassSWSta_flg"
  [VHAL_CSW2PassSWSta_flg] -> UnitConverter274/1
  Shifter2/7(VHAL_CSW2RWipWasSwSta_enum) -> [VHAL_CSW2RWipWasSwSta_enum]
  UnitConverter275/1 -> bus_creator/297  "VHAL_CSW2RWipWasSwSta_enum"
  [VHAL_CSW2RWipWasSwSta_enum] -> UnitConverter275/1
  Shifter2/8(VHAL_CSW2TurnSwSta_enum) -> [VHAL_CSW2TurnSwSta_enum]
  UnitConverter276/1 -> bus_creator/298  "VHAL_CSW2TurnSwSta_enum"
  [VHAL_CSW2TurnSwSta_enum] -> UnitConverter276/1
